simulink model "GFM_29bus"  (R2018b)
settings: Solver=ode1  StartTime=0.0  StopTime=4.5  FixedStep=Time_Step  RelTol=1e-3  EnableMultiTasking=on
PreLoadFcn:
  | Init_29bus;
InitFcn:
  | Init_29bus;
undefined symbols (not defined in the file): D1, D11, Delta, Time_Step, VSC01_Delta_P_Time_Step, VSC01_Delta_P_Value
libraries: powerlib x175, GFM_Lib x1
(part 2 of 5)

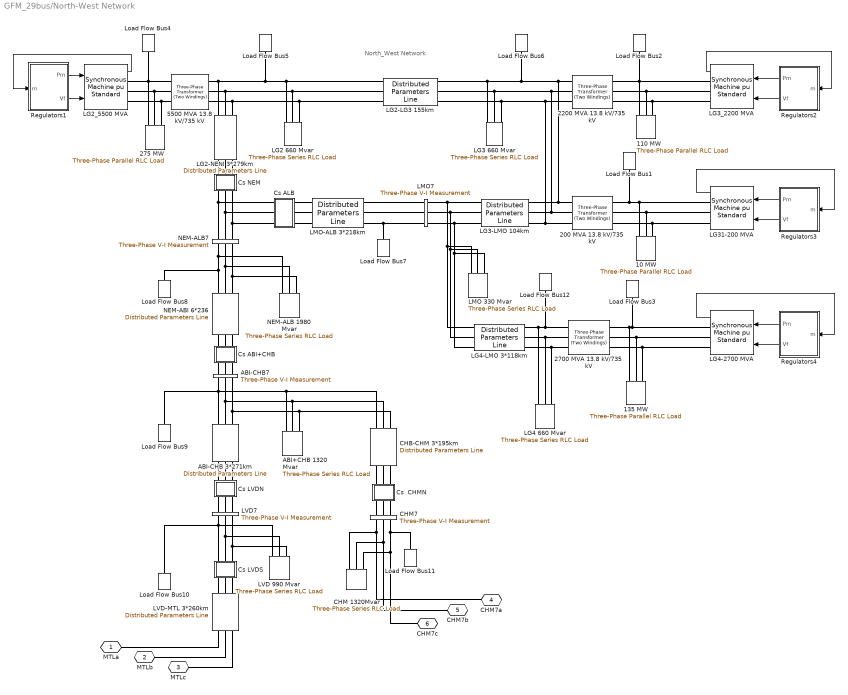
== system GFM_29bus/North-West Network ==
  note: North_West Network
  10 MW : powerlib/Elements/Three-Phase Parallel RLC Load  LConnTagsString=A|B|C  Configuration=Y (grounded)  NominalVoltage=(13800)*1  Vabc=[1e3 1e3 1e3]  Vabcp=[1e3 1e3 1e3]  NominalFrequency=60  UnbalancedPower=off  ActivePower=10000000  InductivePower=0  CapacitivePower=0  Pabc=[10e3 9e3 11e3]  QLabc=[100 90 110]  QCabc=[100 90 110]  Pabcp=[10e3 9e3 11e3]  QLabcp=[100 90 110]  QCabcp=[100 90 110]  Measurements=None  LoadType=constant PQ
  110 MW : powerlib/Elements/Three-Phase Parallel RLC Load  LConnTagsString=A|B|C  Configuration=Y (grounded)  NominalVoltage=(13800)*1  Vabc=[1e3 1e3 1e3]  Vabcp=[1e3 1e3 1e3]  NominalFrequency=60  UnbalancedPower=off  ActivePower=110000000  InductivePower=0  CapacitivePower=0  Pabc=[10e3 9e3 11e3]  QLabc=[100 90 110]  QCabc=[100 90 110]  Pabcp=[10e3 9e3 11e3]  QLabcp=[100 90 110]  QCabcp=[100 90 110]  Measurements=None  LoadType=constant PQ
  135 MW : powerlib/Elements/Three-Phase Parallel RLC Load  LConnTagsString=A|B|C  Configuration=Y (grounded)  NominalVoltage=(13800)*1  Vabc=[1e3 1e3 1e3]  Vabcp=[1e3 1e3 1e3]  NominalFrequency=60  UnbalancedPower=off  ActivePower=135000000  InductivePower=0  CapacitivePower=0  Pabc=[10e3 9e3 11e3]  QLabc=[100 90 110]  QCabc=[100 90 110]  Pabcp=[10e3 9e3 11e3]  QLabcp=[100 90 110]  QCabcp=[100 90 110]  Measurements=None  LoadType=constant PQ
  200 MVA 13.8 kV/735 kV : powerlib/Elements/Three-Phase Transformer (Two Windings)  Winding1Connection=Delta (D1)  Winding2Connection=Yg  CoreType=Three single-phase transformers  SetSaturation=off  Hysteresis=off  DataFile='basic_model'  SetInitialFlux=off  Measurements=None  UNITS=pu  NominalPower=[ 200e6 60 ]  Winding1="[ 13.8e3 0.002  0.0]"  Winding2=[ 735e3 0.002 0.12]  Rm=500  Lm=500  L0=0.5  Saturation="[ 0,0  ;  0.005,1.2  ;  1.0,1.4 ]"  InitialFluxes=[ 0.8 , -0.8 , 0.7 ]  BreakLoop=off  DiscreteSolver=Trapezoidal iterative  DataType=off  TransfoNumber=0
  2200 MVA 13.8 kV/735 kV : powerlib/Elements/Three-Phase Transformer (Two Windings)  Winding1Connection=Delta (D1)  Winding2Connection=Yg  CoreType=Three single-phase transformers  SetSaturation=off  Hysteresis=off  DataFile='basic_model'  SetInitialFlux=off  Measurements=None  UNITS=pu  NominalPower=[ 2200e6 60 ]  Winding1="[ 13.8e3 0.002  0.0]"  Winding2=[ 735e3 0.002 0.12]  Rm=500  Lm=500  L0=0.5  Saturation="[ 0,0  ;  0.005,1.2  ;  1.0,1.4 ]"  InitialFluxes=[ 0.8 , -0.8 , 0.7 ]  BreakLoop=off  DiscreteSolver=Trapezoidal iterative  DataType=off  TransfoNumber=0
  2700 MVA 13.8 kV/735 kV : powerlib/Elements/Three-Phase Transformer (Two Windings)  Winding1Connection=Delta (D1)  Winding2Connection=Yg  CoreType=Three single-phase transformers  SetSaturation=off  Hysteresis=off  DataFile='basic_model'  SetInitialFlux=off  Measurements=None  UNITS=pu  NominalPower=[ 2700e6 60 ]  Winding1="[ 13.8e3 0.002  0.0]"  Winding2=[ 735e3 0.002 0.12]  Rm=500  Lm=500  L0=0.5  Saturation="[ 0,0  ;  0.005,1.2  ;  1.0,1.4 ]"  InitialFluxes=[ 0.8 , -0.8 , 0.7 ]  BreakLoop=off  DiscreteSolver=Trapezoidal iterative  DataType=off  TransfoNumber=0
  275 MW : powerlib/Elements/Three-Phase Parallel RLC Load  LConnTagsString=A|B|C  Configuration=Y (grounded)  NominalVoltage=(13800)*1  Vabc=[1e3 1e3 1e3]  Vabcp=[1e3 1e3 1e3]  NominalFrequency=60  UnbalancedPower=off  ActivePower=275000000  InductivePower=0  CapacitivePower=0  Pabc=[10e3 9e3 11e3]  QLabc=[100 90 110]  QCabc=[100 90 110]  Pabcp=[10e3 9e3 11e3]  QLabcp=[100 90 110]  QCabcp=[100 90 110]  Measurements=None  LoadType=constant PQ
  5500 MVA 13.8 kV/735 kV : powerlib/Elements/Three-Phase Transformer (Two Windings)  Winding1Connection=Delta (D1)  Winding2Connection=Yg  CoreType=Three single-phase transformers  SetSaturation=off  Hysteresis=off  DataFile='basic_model'  SetInitialFlux=off  Measurements=None  UNITS=pu  NominalPower=[ 5500e6 60 ]  Winding1="[ 13.8e3 0.002  0.0]"  Winding2=[ 735e3 0.002 0.12]  Rm=500  Lm=500  L0=0.5  Saturation="[ 0,0  ;  0.005,1.2  ;  1.0,1.4 ]"  InitialFluxes=[ 0.8 , -0.8 , 0.7 ]  BreakLoop=off  DiscreteSolver=Trapezoidal iterative  DataType=off  TransfoNumber=0
  ABI+CHB 1320 Mvar : powerlib/Elements/Three-Phase Series RLC Load  LConnTagsString=A|B|C  Configuration=Y (grounded)  NominalVoltage=735e3  Vabc=[1e3 1e3 1e3]  Vabcp=[1e3 1e3 1e3]  NominalFrequency=60  UnbalancedPower=off  ActivePower=4400000  InductivePower=1320e6  CapacitivePower=0  Pabc=[10e3 9e3 11e3]  QLabc=[100 90 110]  QCabc=[100 90 110]  Pabcp=[10e3 9e3 11e3]  QLabcp=[100 90 110]  QCabcp=[100 90 110]  Measurements=None  LoadType=constant Z
  ABI-CHB 3*271km : powerlib/Elements/Distributed Parameters Line  Phases=3  Length=271  Frequency=60  Resistance="[0.01273  0.3864]/3"  Inductance="[0.9337e-3  4.1264e-3]/3"  Capacitance=[12.74e-9 7.751e-9]*3  x1=[-0.00156 -3.96687684446933e-08 0 0;-0.00152 -3.91975334867025e-08 0 0;-0.00148 -3.87173853476219e-08 0 0;-0.00144 -3.82284332089978e-08 0 0;-0.0014 -3.773078825433e-08 0 0;-0.00136 -3.72245636437896e-08 0 0;-0.00132 -3.67098744884875e-08 0 0;-0.00128 -3.61868378242992e-08 0 0;-0.00124 -3.56555725852517e-08 0 0;-0.0012 -3.51161995764789e-08 0 0;-0.00116 -3.45688414467516e-08 0 0;-0.00112 -3.40136226605882e-08 0 0;-0.00108 -3.34506694699529e-08 0 0;-0.00104 -3.28801098855464e-08 0 0;-0.001 -3.23020736476978e-08 0 0;-0.00096 -3.17166921968631e-08 187821.103557323 -755234.225715977;-0.00092 -3.11240986437358e-08 199188.008257712 -752316.171268998;-0.00088 -3.05244277389798e-08 210509.619322748 -749227.046612372;-0.00084 -2.99178158425874e-08 221783.362315707 -745967.554186405;-0.0008 -2.93044008928726e-08 233006.673684654 -742538.435171566;-0.00076 -2.86843223751052e-08 244177.00134537 -738940.469319947;-0.00072 -2.80577212897927e-08 255291.805261672 -735174.474777957;-0.00068 -2.74247401206185e-08 266348.558023 -731241.307900276;-0.00064 -2.67855228020416e-08 277344.745419126 -727141.863055136;-0.0006 -2.61402146865681e-08 288277.867011863 -722877.072420941;-0.00056 -2.54889625116985e-08 299145.436703644 -718447.905774304;-0.00052 -2.48319143665612e-08 309944.983302838 -713855.370269525;-0.00048 -2.41692196582383e-08 320674.051085682 -709100.510209573;-0.00044 -2.35010290777915e-08 331330.200354684 -704184.406808622;-0.0004 -2.28274945659967e-08 341911.007993395 -699108.17794619;-0.00036 -2.21487692787935e-08 352414.068017403 -693872.977912945;-0.00032 -2.14650075524591e-08 362836.992121434 -688479.997148229;-0.00028 -2.07763648685137e-08 373177.410222429 -682930.46196936;-0.00024 -2.00829978183649e-08 383432.970998484 -677225.63429278;-0.0002 -1.93850640677006e-08 393601.34242352 -671366.811347108;-0.00016 -1.8682722320637e-08 403680.212297562 -665355.325378155;-0.00012 -1.79761322836306e-08 413667.288772517 -659192.543345992;-8e-05 -1.72654546291625e-08 423560.300873321 -652879.866614107;-4e-05 -1.65508509592027e-08 433356.999014334 -646418.730630749]  x2=[-0.00156 -8.24539782860375e-08 0 0;-0.00152 -8.14137848863291e-08 0 0;-0.00148 -8.03550786940201e-08 0 0;-0.00144 -7.92781004497688e-08 0 0;-0.0014 -7.81830950491404e-08 0 0;-0.00136 -7.70703114869202e-08 0 0;-0.00132 -7.59400028004939e-08 0 0;-0.00128 -7.47924260123094e-08 0 0;-0.00124 -7.36278420714322e-08 0 0;-0.0012 -7.24465157942074e-08 0 0;-0.00116 -7.12487158040431e-08 0 0;-0.00112 -7.00347144703277e-08 0 0;-0.00108 -6.88047878464955e-08 0 0;-0.00104 -6.75592156072541e-08 0 0;-0.001 -6.62982809849896e-08 0 0;-0.00096 -6.50222707053611e-08 -41956.1732739779 -761002.997662075;-0.00092 -6.37314749221023e-08 -30476.1660907915 -761549.111628015;-0.00088 -6.24261871510431e-08 -18989.2288902512 -761922.055893291;-0.00084 -6.11067042033663e-08 -7497.97370281746 -762121.745653593;-0.0008 -5.97733261181154e-08 3994.98645917652 -762148.135501191;-0.00076 -5.84263560939685e-08 15487.0381957011 -762001.219435262;-0.00072 -5.70661004202932e-08 26975.5683132944 -761681.030863252;-0.00068 -5.56928684074994e-08 38457.9644192806 -761187.642593282;-0.00064 -5.43069723167046e-08 49931.6155158053 -760521.166817588;-0.0006 -5.29087272887284e-08 61393.9125935536 -759681.755087015;-0.00056 -5.14984512724322e-08 72842.2492250167 -758669.598276551;-0.00052 -5.00764649524203e-08 84274.0221571708 -757484.926541928;-0.00048 -4.86430916761193e-08 95686.6319034346 -756128.00926728;-0.00044 -4.71986573802513e-08 107077.48333477 -754599.155003896;-0.0004 -4.57434905167189e-08 118443.986269792 -752898.71140005;-0.00036 -4.42779219779181e-08 129783.556063753 -751027.065121953;-0.00032 -4.2802285021496e-08 141093.614196272 -748984.641765829;-0.00028 -4.13169151945712e-08 152371.588857661 -746771.905761136;-0.00024 -3.98221502574331e-08 163614.915533741 -744389.360264959;-0.0002 -3.83183301067381e-08 174821.037588984 -741837.547047599;-0.00016 -3.680579669822e-08 185987.406847871 -739117.046369375;-0.00012 -3.52848939689323e-08 197111.484174328 -736228.47684868;-8e-05 -3.37559677590401e-08 208190.740049101 -733172.495321314;-4e-05 -3.22193657331786e-08 219222.655144948 -729949.796691121]  x3=[-0.00156 -4.97060323713084e-10 0 0;-0.00152 -4.99355267685027e-10 0 0;-0.00148 -5.01536662575356e-10 0 0;-0.00144 -5.03604012353683e-10 0 0;-0.0014 -5.05556846922497e-10 0 0;-0.00136 -5.07394722224057e-10 0 0;-0.00132 -5.09117220341369e-10 0 0;-0.00128 -5.10723949593215e-10 0 0;-0.00124 -5.1221454462322e-10 0 0;-0.0012 -5.13588666482928e-10 0 0;-0.00116 -5.14846002708877e-10 0 0;-0.00112 -5.15986267393653e-10 0 0;-0.00108 -5.170092012509e-10 0 0;-0.00104 -5.1791457167428e-10 0 0;-0.001 -5.18702172790366e-10 0 0;-0.00096 -5.19371825505456e-10 139.184757397711 -1341.52529810437;-0.00092 -5.19923377546299e-10 159.398007251781 -1339.2740416806;-0.00088 -5.20356703494716e-10 179.575011373592 -1336.71824588915;-0.00084 -5.20671704816123e-10 199.711181686405 -1333.85849189596;-0.0008 -5.20868309881937e-10 219.801939398739 -1330.69542998441;-0.00076 -5.2094647398586e-10 239.842716045545 -1327.22977940752;-0.00072 -5.2090617935405e-10 259.828954527038 -1323.46232822433;-0.00068 -5.20747435149159e-10 279.75611014494 -1319.39393312075;-0.00064 -5.20470277468249e-10 299.61965163591 -1315.02551921475;-0.0006 -5.20074769334587e-10 319.415062201907 -1310.35807984598;-0.00056 -5.19561000683313e-10 339.137840537278 -1305.3926763499;-0.00052 -5.18929088340986e-10 358.783501852311 -1300.13043781644;-0.00048 -5.18179175999025e-10 378.34757889304 -1294.57256083327;-0.00044 -5.17311434181028e-10 397.825622957059 -1288.72030921369;-0.0004 -5.16326060204003e-10 417.213204905119 -1282.57501370924;-0.00036 -5.15223278133493e-10 436.505916168278 -1276.13807170713;-0.00032 -5.14003338732632e-10 455.699369750367 -1269.41094691246;-0.00028 -5.12666519405119e-10 474.789201225558 -1262.3951690154;-0.00024 -5.11213124132141e-10 493.771069730799 -1255.09233334333;-0.0002 -5.0964348340325e-10 512.640658952883 -1247.50410049812;-0.00016 -5.07957954141212e-10 531.393678109946 -1239.63219597847;-0.00012 -5.06156919620844e-10 550.02586292715 -1231.47840978759;-8e-05 -5.04240789381866e-10 568.532976606346 -1223.04459602614;-4e-05 -5.0220999913577e-10 586.910810789482 -1214.33267247064]  x4=[-0.00156 -7.23499245139953e-11 0 0;-0.00152 -6.66102552922797e-11 0 0;-0.00148 -6.08554394729331e-11 0 0;-0.00144 -5.50867856514452e-11 0 0;-0.0014 -4.93056055699484e-11 0 0;-0.00136 -4.35132138189384e-11 0 0;-0.00132 -3.7710927538348e-11 0 0;-0.00128 -3.19000661180405e-11 0 0;-0.00124 -2.60819508977922e-11 0 0;-0.0012 -2.0257904866831e-11 0 0;-0.00116 -1.44292523629998e-11 0 0;-0.00112 -8.59731877161376e-12 0 0;-0.00108 -2.76343022407925e-12 0 0;-0.00104 3.07108670365746e-12 0 0;-0.001 8.90490529276171e-12 0 0;-0.00096 1.4736698983195e-11 -1510.56660851053 -15585.3215951668;-0.00092 2.05651416753633e-11 -1275.38237576371 -15606.3269526567;-0.00088 2.63889080316609e-11 -1039.90813206307 -15623.7835659808;-0.00084 3.22066737778404e-11 -804.197422220979 -15637.6874656559;-0.0008 3.80171160041413e-11 -568.303844820181 -15648.0354900548;-0.00076 4.38189134661086e-11 -332.281040025915 -15654.8252861263;-0.00072 4.96107468850318e-11 -96.1826773886164 -15658.0553099292;-0.00068 5.53912992479382e-11 139.937556360077 -15657.7248269839;-0.00064 6.11592561070699e-11 376.025969515224 -15653.8339124394;-0.0006 6.69133058787778e-11 612.028877607613 -15646.3834510561;-0.00056 7.26521401417647e-11 847.892615611145 -15635.3751370047;-0.00052 7.83744539346086e-11 1083.5635501458 -15620.8114734809;-0.00048 8.40789460525004e-11 1318.98809167341 -15602.6957721362;-0.00044 8.97643193431258e-11 1554.11270668344 -15581.0321523248;-0.0004 9.5429281001627e-11 1788.88392986607 -15555.8255401671;-0.00036 1.01072542864576e-10 2023.24837626972 -15527.0816674293;-0.00032 1.06692821702889e-10 2257.15275344037 -15494.8070702201;-0.00028 1.12288839513627e-10 2490.54387353973 -15459.0090875047;-0.00024 1.17859323810598e-10 2723.36866543979 -15419.6958594356;-0.0002 1.23403007913709e-10 2955.57418679066 -15376.8763255019;-0.00016 1.28918631237003e-10 3187.10763605924 -15330.5602224963;-0.00012 1.34404939575301e-10 3417.91636453582 -15280.7580823012;-8e-05 1.39860685389398e-10 3647.94788830597 -15227.4812294938;-4e-05 1.45284628089745e-10 3877.14990018487 -15170.7417787711]  x5=0.00153261764655846  V1=ones(3,3)  V2=ones(3,3)  I1=ones(3,3)  I2=ones(3,3)  nHarmo=1  Measurements=None  Decoupling=off  VsMag0=0  VrMag0=0  VsAngle0=0  VrAngle0=0  IsMag0=0  IrMag0=0  IsAngle0=0  IrAngle0=0
      settings: AttributesFormatString=\n
  ABI-CHB7 : powerlib/Measurements/Three-Phase V-I Measurement  VoltageMeasurement=no  SetLabelV=on  LabelV=Vabc_ABI7  Vpu=on  VpuLL=off  CurrentMeasurement=no  SetLabelI=off  LabelI=A1  Ipu=off  Pbase=100e6  Vbase=500e3  OutputType=Magnitude  PhasorSimulation=off  PSBequivalent=0
  CHB-CHM 3*195km : powerlib/Elements/Distributed Parameters Line  Phases=3  Length=195  Frequency=60  Resistance="[0.01273  0.3864]/3"  Inductance="[0.9337e-3  4.1264e-3]/3"  Capacitance=[12.74e-9 7.751e-9]*3  x1=[-0.00112 -3.40136226605882e-08 0 0;-0.00108 -3.34506694699529e-08 0 0;-0.00104 -3.28801098855464e-08 0 0;-0.001 -3.23020736476978e-08 0 0;-0.00096 -3.17166921968631e-08 0 0;-0.00092 -3.11240986437358e-08 0 0;-0.00088 -3.05244277389798e-08 0 0;-0.00084 -2.99178158425874e-08 0 0;-0.0008 -2.93044008928726e-08 0 0;-0.00076 -2.86843223751052e-08 0 0;-0.00072 -2.80577212897927e-08 0 0;-0.00068 -2.74247401206185e-08 266348.558023 -731241.307900276;-0.00064 -2.67855228020416e-08 277344.745419126 -727141.863055136;-0.0006 -2.61402146865681e-08 288277.867011863 -722877.072420941;-0.00056 -2.54889625116985e-08 299145.436703644 -718447.905774304;-0.00052 -2.48319143665612e-08 309944.983302838 -713855.370269525;-0.00048 -2.41692196582383e-08 320674.051085682 -709100.510209573;-0.00044 -2.35010290777915e-08 331330.200354684 -704184.406808622;-0.0004 -2.28274945659967e-08 341911.007993395 -699108.17794619;-0.00036 -2.21487692787935e-08 352414.068017403 -693872.977912945;-0.00032 -2.14650075524591e-08 362836.992121434 -688479.997148229;-0.00028 -2.07763648685137e-08 373177.410222429 -682930.46196936;-0.00024 -2.00829978183649e-08 383432.970998484 -677225.63429278;-0.0002 -1.93850640677006e-08 393601.34242352 -671366.811347108;-0.00016 -1.8682722320637e-08 403680.212297562 -665355.325378155;-0.00012 -1.79761322836306e-08 413667.288772517 -659192.543345992;-8e-05 -1.72654546291625e-08 423560.300873321 -652879.866614107;-4e-05 -1.65508509592027e-08 433356.999014334 -646418.730630749]  x2=[-0.00112 -2.2052791971615e-08 0 0;-0.00108 -2.16420683624788e-08 0 0;-0.00104 -2.12264235336303e-08 0 0;-0.001 -2.08059519991191e-08 0 0;-0.00096 -2.03807493705462e-08 0 0;-0.00092 -1.99509123353226e-08 0 0;-0.00088 -1.95165386346832e-08 0 0;-0.00084 -1.90777270414618e-08 0 0;-0.0008 -1.86345773376304e-08 0 0;-0.00076 -1.81871902916102e-08 0 0;-0.00072 -1.77356676353574e-08 0 0;-0.00068 -1.72801120412301e-08 189054.242567797 -739105.585396465;-0.00064 -1.68206270986421e-08 200177.800883661 -736170.765273225;-0.0006 -1.63573172905067e-08 211255.840493863 -733068.546266429;-0.00056 -1.58902879694789e-08 222285.84234773 -729799.633793925;-0.00052 -1.54196453339989e-08 233265.298317959 -726364.771178221;-0.00048 -1.49454964041433e-08 244191.711770944 -722764.739477454;-0.00044 -1.44679489972898e-08 255062.598134493 -719000.357307787;-0.0004 -1.39871117036007e-08 265875.485462792 -715072.480657264;-0.00036 -1.35030938613299e-08 276627.914998509 -710982.002691161;-0.00032 -1.30160055319607e-08 287317.441731892 -706729.853548894;-0.00028 -1.25259574751788e-08 297941.634956747 -702317.000132509;-0.00024 -1.20330611236863e-08 308498.078823151 -697744.445886818;-0.0002 -1.1537428557863e-08 318984.372886805 -693013.230571223;-0.00016 -1.10391724802802e-08 329398.132654868 -688124.430023288;-0.00012 -1.05384061900731e-08 339736.990128175 -683079.155914099;-8e-05 -1.00352435571778e-08 349998.594339693 -677878.555495478;-4e-05 -9.52979899643775e-09 360180.611889118 -672523.811339114]  x3=[-0.00112 -4.51346938208632e-11 0 0;-0.00108 -4.21049821896206e-11 0 0;-0.00104 -3.90656962485261e-11 0 0;-0.001 -3.60175271049928e-11 0 0;-0.00096 -3.29611678863978e-11 0 0;-0.00092 -2.98973135824704e-11 0 0;-0.00088 -2.68266608872578e-11 0 0;-0.00084 -2.37499080407027e-11 0 0;-0.0008 -2.06677546698697e-11 0 0;-0.00076 -1.75809016298559e-11 0 0;-0.00072 -1.44900508444226e-11 0 0;-0.00068 -1.13959051463842e-11 1436.63532489199 -5039.5712074965;-0.00064 -8.29916811778968e-12 1512.46399636275 -5017.33500426099;-0.0006 -5.2005439299341e-12 1587.94874656368 -4993.95790231317;-0.00056 -2.10073718323644e-12 1663.07241091352 -4969.44521740442;-0.00052 9.99547252980699e-13 1737.81790693885 -4943.8025235079;-0.00048 4.09960440077225e-12 1812.16823815844 -4917.03565155107;-0.00044 7.19872933387654e-12 1886.10649794815 -4889.15068808979;-0.0004 1.02962173380095e-11 1959.61587338531 -4860.15397392427;-0.00036 1.33913640711106e-11 2032.67964907188 -4830.05210265727;-0.00032 1.64834657235041e-11 2105.28121093533 -4798.85191919472;-0.00028 1.95718191779395e-11 2177.40405000658 -4766.56051818929;-0.00024 2.2655722169474e-11 2249.031766174 -4733.18524242708;-0.0002 2.57344734451617e-11 2320.14807191261 -4698.73368115799;-0.00016 2.88073729235127e-11 2390.73679598777 -4663.21366836997;-0.00012 3.18737218536851e-11 2460.78188713236 -4626.6332810076;-8e-05 3.49328229743752e-11 2530.2674176967 -4589.00083713551;-4e-05 3.79839806723688e-11 2599.17758727035 -4550.32489404692]  x4=[-0.00112 -2.24971038730357e-10 0 0;-0.00108 -2.24970289807423e-10 0 0;-0.00104 -2.24918384580647e-10 0 0;-0.001 -2.24815334852831e-10 0 0;-0.00096 -2.24661164056595e-10 0 0;-0.00092 -2.24455907249047e-10 0 0;-0.00088 -2.24199611103816e-10 0 0;-0.00084 -2.23892333900435e-10 0 0;-0.0008 -2.23534145511091e-10 0 0;-0.00076 -2.23125127384734e-10 0 0;-0.00072 -2.22665372528558e-10 0 0;-0.00068 -2.22154985486854e-10 1507.95089400206 -11782.2652584688;-0.00064 -2.21594082317234e-10 1685.44568306095 -11758.1867357336;-0.0006 -2.2098279056424e-10 1862.55721630617 -11731.4345027329;-0.00056 -2.20321249230347e-10 2039.24522010242 -11702.0146426938;-0.00052 -2.19609608744348e-10 2215.46951712132 -11669.9338454389;-0.00048 -2.18848030927153e-10 2391.19003547742 -11635.1994058648;-0.00044 -2.1803668895499e-10 2566.36681784019 -11597.8192222834;-0.0004 -2.17175767320028e-10 2740.96003052 -11557.8017946263;-0.00036 -2.1626546178842e-10 2914.9299725259 -11515.1562225112;-0.00032 -2.15305979355796e-10 3088.23708459333 -11469.8922031737;-0.00028 -2.14297538200187e-10 3260.84195817954 -11422.0200292613;-0.00024 -2.13240367632413e-10 3432.70534442477 -11371.5505864935;-0.0002 -2.12134708043947e-10 3603.78816307707 -11318.4953511865;-0.00016 -2.10980810852243e-10 3774.05151137883 -11262.8663876431;-0.00012 -2.09778938443573e-10 3943.45667291294 -11204.67634541;-8e-05 -2.08529364113357e-10 4111.96512640654 -11143.938456401;-4e-05 -2.07232372004022e-10 4279.53855449048 -11080.6665318882]  x5=0.0011028060556417  V1=ones(3,3)  V2=ones(3,3)  I1=ones(3,3)  I2=ones(3,3)  nHarmo=1  Measurements=None  Decoupling=off  VsMag0=0  VrMag0=0  VsAngle0=0  VrAngle0=0  IsMag0=0  IrMag0=0  IsAngle0=0  IrAngle0=0
      settings: AttributesFormatString=\n
  CHM 1320Mvar : powerlib/Elements/Three-Phase Series RLC Load  LConnTagsString=A|B|C  Configuration=Y (grounded)  NominalVoltage=735e3  Vabc=[1e3 1e3 1e3]  Vabcp=[1e3 1e3 1e3]  NominalFrequency=60  UnbalancedPower=off  ActivePower=4400000  InductivePower=1320e6  CapacitivePower=0  Pabc=[10e3 9e3 11e3]  QLabc=[100 90 110]  QCabc=[100 90 110]  Pabcp=[10e3 9e3 11e3]  QLabcp=[100 90 110]  QCabcp=[100 90 110]  Measurements=None  LoadType=constant Z
  CHM7 : powerlib/Measurements/Three-Phase V-I Measurement  VoltageMeasurement=no  SetLabelV=on  LabelV=Vabc_CHM7  Vpu=on  VpuLL=off  CurrentMeasurement=no  SetLabelI=off  LabelI=A1  Ipu=off  Pbase=100e6  Vbase=735e3  OutputType=Magnitude  PhasorSimulation=off  PSBequivalent=0
  "Cs  CHMN " : Subsystem  mask{Xc=25/3}
      mask prompts: Xc "Condensator Reactance at  60Hz  (ohm):"
      mask help: Series Compensation
      mask init:
      | Cs=1/Xc/(2*pi*60);
      mask Display: disp('Cs')
  "Cs ABI+CHB " : Subsystem  mask{Xc=25/6}
      mask prompts: Xc "Condensator Reactance at  60Hz  (ohm):"
      mask help: Series Compensation
      mask init:
      | Cs=1/Xc/(2*pi*60);
      mask Display: disp('Cs')
  Cs ALB : Subsystem  mask{Xc=16/3}
      mask prompts: Xc "Reactance @ 60Hz du condensateur (ohm):"
      mask init:
      | Cs=1/Xc/(2*pi*60);
      mask Display: disp('Cs')
  "Cs LVDN " : Subsystem  mask{Xc=34/3}
      mask prompts: Xc "Condensator Reactance at  60Hz  (ohm):"
      mask help: Series Compensation
      mask init:
      | Cs=1/Xc/(2*pi*60);
      mask Display: disp('Cs')
  "Cs LVDS " : Subsystem  mask{Xc=34/3}
      mask prompts: Xc "Condensator Reactance at  60Hz  (ohm):"
      mask help: Series Compensation
      mask init:
      | Cs=1/Xc/(2*pi*60);
      mask Display: disp('Cs')
  "Cs NEM " : Subsystem  mask{Xc=16/3}
      mask prompts: Xc "Condensator Reactance at  60Hz  (ohm):"
      mask help: Series Compensation
      mask init:
      | Cs=1/Xc/(2*pi*60);
      mask Display: disp('Cs')
  LG2 660 Mvar : powerlib/Elements/Three-Phase Series RLC Load  LConnTagsString=A|B|C  Configuration=Y (grounded)  NominalVoltage=735e3  Vabc=[1e3 1e3 1e3]  Vabcp=[1e3 1e3 1e3]  NominalFrequency=60  UnbalancedPower=off  ActivePower=2200000  InductivePower=660e6  CapacitivePower=0  Pabc=[10e3 9e3 11e3]  QLabc=[100 90 110]  QCabc=[100 90 110]  Pabcp=[10e3 9e3 11e3]  QLabcp=[100 90 110]  QCabcp=[100 90 110]  Measurements=None  LoadType=constant Z
  LG2-LG3 155km : powerlib/Elements/Distributed Parameters Line  Phases=3  Length=155  Frequency=60  Resistance="[0.01273  0.3864]"  Inductance="[0.9337e-3  4.1264e-3]"  Capacitance=[12.74e-9 7.751e-9]  x1=[-0.00088 -2.46870498089306e-09 432967.319119817 -601760.567731855;-0.00084 -2.4236910908169e-09 441992.1177872 -595163.398551982;-0.0008 -2.37812607428771e-09 450916.411258577 -588430.89434775;-0.00076 -2.33202029239731e-09 459738.17022657 -581564.586032555;-0.00072 -2.28538422920291e-09 468455.388699268 -574566.034945695;-0.00068 -2.2382284893431e-09 477066.084456362 -567436.832497335;-0.00064 -2.19056379562648e-09 485568.299499894 -560178.599806632;-0.0006 -2.14240098659334e-09 493960.100499482 -552792.987333108;-0.00056 -2.09375101405114e-09 502239.579231947 -545281.674501348;-0.00052 -2.04462494058408e-09 510404.853015224 -537646.369319115;-0.00048 -1.99503393703763e-09 518454.06513647 -529888.807988964;-0.00044 -1.94498927997833e-09 526385.385274261 -522010.754513442;-0.0004 -1.89450234912964e-09 534197.009914795 -514014.000293973;-0.00036 -1.84358462478425e-09 541887.162761993 -505900.363723505;-0.00032 -1.79224768519358e-09 549454.095141415 -497671.689773026;-0.00028 -1.74050320393498e-09 556896.086397892 -489329.84957203;-0.00024 -1.68836294725727e-09 564211.44428679 -480876.739983042;-0.0002 -1.63583877140518e-09 571398.505358808 -472314.283170286;-0.00016 -1.58294261992334e-09 578455.63533824 -463644.426162603;-0.00012 -1.52968652094044e-09 585381.229494584 -454869.140410709;-8e-05 -1.47608258443414e-09 592173.713007454 -445990.42133891;-4e-05 -1.42214299947733e-09 598831.541324674 -437010.287891357]  x2=[-0.00088 -9.77818774096488e-10 445023.73878971 -584526.591412552;-0.00084 -9.6050679070525e-10 453787.292631294 -577749.57858463;-0.0008 -9.42976396352864e-10 462447.659155828 -570841.190484839;-0.00076 -9.2523157729983e-10 471002.869070649 -563802.998021056;-0.00072 -9.07276368564974e-10 479450.976994799 -556636.601617554;-0.00068 -8.89114853007925e-10 487790.061901389 -549343.630851073;-0.00064 -8.70751160400702e-10 496018.227554425 -541925.744080274;-0.0006 -8.52189466488643e-10 504133.602939995 -534384.62806864;-0.00056 -8.33433992040872e-10 512134.342691719 -526721.99760092;-0.00052 -8.1448900189054e-10 520018.627510373 -518939.595093203;-0.00048 -7.95358803965032e-10 527784.664577582 -511039.190196705;-0.00044 -7.76047748306385e-10 535430.687963486 -503022.579395372;-0.0004 -7.56560226082124e-10 542954.959028305 -494891.585597366;-0.00036 -7.36900668586749e-10 550355.766817685 -486648.057720558;-0.00032 -7.17073546234098e-10 557631.428451757 -478293.870272098;-0.00028 -6.97083367540812e-10 564780.289507808 -469830.92292217;-0.00024 -6.76934678101139e-10 571800.724396482 -461261.140072018;-0.0002 -6.56632059553301e-10 578691.136731428 -452586.470416361;-0.00016 -6.36180128537675e-10 585449.959692301 -443808.88650027;-0.00012 -6.15583535647003e-10 592075.656381045 -434930.384270634;-8e-05 -5.94846964368891e-10 598566.720171371 -425952.982622295;-4e-05 -5.73975130020824e-10 604921.67505135 -416878.72293897]  x3=[-0.00088 4.31670369824933e-12 1691.04104798713 -2581.82778924969;-0.00084 4.4152064901244e-12 1729.78041093162 -2556.03490983374;-0.0008 4.51270530211874e-12 1768.12643672765 -2529.66081012159;-0.00076 4.60917796384329e-12 1806.07040581965 -2502.71148735608;-0.00072 4.70460253824672e-12 1843.60369007625 -2475.19306958082;-0.00068 4.79895732660372e-12 1880.71775475228 -2447.11181424669;-0.00064 4.89222087344909e-12 1917.40416042951 -2418.47410678899;-0.0006 4.98437197145656e-12 1953.65456493564 -2389.28645917544;-0.00056 5.07538966626111e-12 1989.4607252413 -2359.55550842541;-0.00052 5.16525326122385e-12 2024.81449933443 -2329.2880151007;-0.00048 5.25394232213823e-12 2059.70784807166 -2298.49086176827;-0.00044 5.34143668187663e-12 2094.1328370064 -2267.17105143523;-0.0004 5.42771644497616e-12 2128.08163819305 -2235.33570595634;-0.00036 5.51276199216273e-12 2161.54653196696 -2202.99206441462;-0.00032 5.59655398481232e-12 2194.51990869988 -2170.14748147526;-0.00028 5.67907336934839e-12 2226.9942705303 -2136.80942571316;-0.00024 5.76030138157451e-12 2258.96223306839 -2102.98547791471;-0.0002 5.84021955094119e-12 2290.41652707513 -2068.68332935396;-0.00016 5.91880970474589e-12 2321.35000011533 -2033.91078004368;-0.00012 5.99605397226537e-12 2351.75561818397 -1998.67573696172;-8e-05 6.07193478881933e-12 2381.62646730571 -1962.98621225302;-4e-05 6.14643489976444e-12 2410.95575510706 -1926.85032140772]  x4=[-0.00088 -1.00528972699252e-11 1092.95151191299 -2102.92038476547;-0.00084 -1.00865716563435e-11 1124.53751640733 -2086.20052208695;-0.0008 -1.011795244335e-11 1155.86781076804 -2069.00627540033;-0.00076 -1.01470324952244e-11 1186.93527075636 -2051.34155452904;-0.00072 -1.01738051994137e-11 1217.7328318998 -2033.21037627826;-0.00068 -1.01982644680358e-11 1248.25349109855 -2014.61686352158;-0.00064 -1.02204047392639e-11 1278.49030821791 -1995.56524426345;-0.0006 -1.02402209785914e-11 1308.4364076664 -1976.05985067779;-0.00056 -1.02577086799762e-11 1338.08497995927 -1956.10511812291;-0.00052 -1.02728638668659e-11 1367.42928326685 -1935.70558413289;-0.00048 -1.02856830931017e-11 1396.46264494762 -1914.86588738586;-0.00044 -1.0296163443702e-11 1425.17846306551 -1893.59076664914;-0.0004 -1.03043025355256e-11 1453.57020789111 -1871.88505970171;-0.00036 -1.03100985178132e-11 1481.6314233865 -1849.75370223415;-0.00032 -1.03135500726083e-11 1509.35572867325 -1827.20172672631;-0.00028 -1.03146564150571e-11 1536.73681948344 -1804.23426130292;-0.00024 -1.0313417293587e-11 1563.76846959312 -1780.85652856756;-0.0002 -1.03098329899634e-11 1590.44453223819 -1757.07384441507;-0.00016 -1.03039043192262e-11 1616.75894151203 -1732.89161682271;-0.00012 -1.02956326295038e-11 1642.70571374491 -1708.31534462051;-8e-05 -1.02850198017072e-11 1668.27894886457 -1683.35061624082;-4e-05 -1.0272068249102e-11 1693.47283173789 -1658.0031084476]  x5=0.000876589428843401  V1=ones(3,3)  V2=ones(3,3)  I1=ones(3,3)  I2=ones(3,3)  nHarmo=1  Measurements=None  Decoupling=off  VsMag0=0  VrMag0=0  VsAngle0=0  VrAngle0=0  IsMag0=0  IrMag0=0  IsAngle0=0  IrAngle0=0
      settings: AttributesFormatString=\n
  LG2-NENI 3*279km : powerlib/Elements/Distributed Parameters Line  Phases=3  Length=279  Frequency=60  Resistance="[0.01273  0.3864]/3"  Inductance="[0.9337e-3  4.1264e-3]/3"  Capacitance=[12.74e-9 7.751e-9]*3  x1=[-0.0016 -3.17369651108322e-09 0 0;-0.00156 -3.14022097034721e-09 0 0;-0.00152 -3.10603137044265e-09 0 0;-0.00148 -3.07113548578973e-09 0 0;-0.00144 -3.03554125141168e-09 0 0;-0.0014 -2.99925676113046e-09 0 0;-0.00136 -2.96229026572624e-09 0 0;-0.00132 -2.9246501710613e-09 0 0;-0.00128 -2.88634503616857e-09 0 0;-0.00124 -2.8473835713054e-09 0 0;-0.0012 -2.80777463597289e-09 0 0;-0.00116 -2.76752723690139e-09 0 0;-0.00112 -2.72665052600236e-09 0 0;-0.00108 -2.68515379828734e-09 0 0;-0.00104 -2.64304648975437e-09 0 0;-0.001 -2.6003381752423e-09 405310.525020648 -620725.219641236;-0.00096 -2.55703856625353e-09 414624.437229961 -614542.931576135;-0.00092 -2.51315750874577e-09 423844.067417816 -608220.901747987;-0.00088 -2.46870498089306e-09 432967.319119817 -601760.567731855;-0.00084 -2.4236910908169e-09 441992.1177872 -595163.398551982;-0.0008 -2.37812607428771e-09 450916.411258577 -588430.89434775;-0.00076 -2.33202029239731e-09 459738.17022657 -581564.586032555;-0.00072 -2.28538422920291e-09 468455.388699268 -574566.034945695;-0.00068 -2.2382284893431e-09 477066.084456362 -567436.832497335;-0.00064 -2.19056379562648e-09 485568.299499894 -560178.599806633;-0.0006 -2.14240098659334e-09 493960.100499482 -552792.987333108;-0.00056 -2.09375101405114e-09 502239.579231947 -545281.674501348;-0.00052 -2.04462494058408e-09 510404.853015224 -537646.369319115;-0.00048 -1.99503393703763e-09 518454.06513647 -529888.807988964;-0.00044 -1.94498927997833e-09 526385.385274261 -522010.754513442;-0.0004 -1.89450234912964e-09 534197.009914795 -514014.000293973;-0.00036 -1.84358462478425e-09 541887.162761993 -505900.363723505;-0.00032 -1.79224768519358e-09 549454.095141415 -497671.689773026;-0.00028 -1.74050320393498e-09 556896.086397892 -489329.84957203;-0.00024 -1.68836294725727e-09 564211.44428679 -480876.739983042;-0.0002 -1.63583877140518e-09 571398.505358808 -472314.283170286;-0.00016 -1.58294261992334e-09 578455.63533824 -463644.426162603;-0.00012 -1.52968652094044e-09 585381.229494584 -454869.140410709;-8e-05 -1.47608258443414e-09 592173.713007454 -445990.42133891;-4e-05 -1.42214299947733e-09 598831.541324674 -437010.287891357]  x2=[-0.0016 -2.46236129996295e-08 0 0;-0.00156 -2.43308871432278e-08 0 0;-0.00152 -2.40326286529104e-08 0 0;-0.00148 -2.37289053500859e-08 0 0;-0.00144 -2.34197862988142e-08 0 0;-0.0014 -2.31053417901017e-08 0 0;-0.00136 -2.27856433259182e-08 0 0;-0.00132 -2.24607636029373e-08 0 0;-0.00128 -2.21307764960066e-08 0 0;-0.00124 -2.17957570413483e-08 0 0;-0.0012 -2.14557814194974e-08 0 0;-0.00116 -2.11109269379785e-08 0 0;-0.00112 -2.07612720137268e-08 0 0;-0.00108 -2.04068961552568e-08 0 0;-0.00104 -2.00478799445826e-08 0 0;-0.001 -1.96843050188946e-08 243857.082602521 -727661.340796743;-0.00096 -1.93162540519955e-08 254801.844915079 -723901.454430001;-0.00092 -1.89438107355012e-08 265688.667485421 -719976.959115181;-0.00088 -1.85670597598102e-08 276515.074743977 -715888.747248675;-0.00084 -1.81860867948453e-08 287278.604859102 -711637.748454607;-0.0008 -1.78009784705734e-08 297976.810296867 -707224.929373443;-0.00076 -1.74118223573064e-08 308607.258377612 -702651.293442187;-0.00072 -1.70187069457885e-08 319167.531829119 -697917.88066621;-0.00068 -1.66217216270741e-08 329655.229336271 -693025.767382756;-0.00064 -1.62209566722015e-08 340067.966087097 -687976.066016199;-0.0006 -1.58165032116651e-08 350403.374315057 -682769.924825083;-0.00056 -1.54084532146941e-08 360659.103837447 -677408.527641018;-0.00052 -1.49968994683389e-08 370832.822589816 -671893.093599491;-0.00048 -1.45819355563724e-08 380922.217156255 -666224.876862638;-0.00044 -1.41636558380096e-08 390924.993295445 -660405.166334065;-0.0004 -1.37421554264515e-08 400838.876462354 -654435.28536576;-0.00036 -1.33175301672566e-08 410661.612325442 -648316.591457172;-0.00032 -1.28898766165472e-08 420390.967279283 -642050.47594653;-0.00028 -1.24592920190528e-08 430024.728952461 -635638.363694466;-0.00024 -1.20258742859976e-08 439560.706710651 -629081.71276001;-0.0002 -1.15897219728364e-08 448996.732154745 -622382.014069042;-0.00016 -1.11509342568442e-08 458330.65961393 -615540.791075268;-0.00012 -1.07096109145635e-08 467560.366633594 -608559.599413801;-8e-05 -1.02658522991166e-08 476683.754457955 -601440.026547423;-4e-05 -9.81975931738582e-09 485698.748507297 -594183.691405605]  x3=[-0.0016 -1.56473012381929e-10 0 0;-0.00156 -1.58154913178634e-10 0 0;-0.00152 -1.59800850911952e-10 0 0;-0.00148 -1.61410451309836e-10 0 0;-0.00144 -1.62983348363037e-10 0 0;-0.0014 -1.64519184408328e-10 0 0;-0.00136 -1.66017610209838e-10 0 0;-0.00132 -1.67478285038462e-10 0 0;-0.00128 -1.68900876749339e-10 0 0;-0.00124 -1.70285061857382e-10 0 0;-0.0012 -1.71630525610834e-10 0 0;-0.00116 -1.72936962062842e-10 0 0;-0.00112 -1.74204074141021e-10 0 0;-0.00108 -1.75431573715012e-10 0 0;-0.00104 -1.76619181661998e-10 0 0;-0.001 -1.77766627930173e-10 -295.521587162754 -2742.85495450109;-0.00096 -1.78873651600151e-10 -254.128191861341 -2746.999265987;-0.00092 -1.79940000944296e-10 -212.677010000606 -2750.51893352893;-0.00088 -1.80965433483962e-10 -171.177467221846 -2753.41315678484;-0.00084 -1.81949716044634e-10 -129.639000163212 -2755.68127763333;-0.0008 -1.82892624808944e-10 -88.0710543138991 -2757.32278032326;-0.00076 -1.83793945367572e-10 -46.4830818663279 -2758.33729159109;-0.00072 -1.84653472767995e-10 -4.88453956679348 -2758.7245807457;-0.00068 -1.85471011561094e-10 36.7151134349161 -2758.48455972087;-0.00064 -1.86246375845597e-10 78.3064177364483 -2757.61728309532;-0.0006 -1.86979389310354e-10 119.879915833873 -2756.12294808028;-0.00056 -1.87669885274424e-10 161.426154272237 -2754.00189447463;-0.00052 -1.88317706724978e-10 202.9356857952 -2751.25460458768;-0.00048 -1.88922706353005e-10 244.399071493256 -2747.88170312946;-0.00044 -1.89484746586808e-10 285.806882950062 -2743.88395706866;-0.0004 -1.90003699623284e-10 327.149704386378 -2739.26227545828;-0.00036 -1.90479447456988e-10 368.418134801137 -2734.01770922885;-0.00032 -1.90911881906965e-10 409.602790109144 -2728.1514509495;-0.00028 -1.9130090464135e-10 450.694305274944 -2721.66483455679;-0.00024 -1.91646427199728e-10 491.683336442347 -2714.55933505133;-0.0002 -1.9194837101325e-10 532.560563059139 -2706.83656816245;-0.00016 -1.92206667422495e-10 573.316689996499 -2698.49828998073;-0.00012 -1.92421257693089e-10 613.942449662625 -2689.54639655873;-8e-05 -1.92592093029053e-10 654.428604110113 -2679.98292347981;-4e-05 -1.92719134583905e-10 694.765947136578 -2669.81004539528]  x4=[-0.0016 2.44847306854454e-11 0 0;-0.00156 2.6808792531249e-11 0 0;-0.00152 2.91267582888202e-11 0 0;-0.00148 3.14381008727351e-11 0 0;-0.00144 3.3742294703622e-11 0 0;-0.0014 3.60388158276746e-11 0 0;-0.00136 3.83271420357934e-11 0 0;-0.00132 4.06067529823325e-11 0 0;-0.00128 4.28771303034211e-11 0 0;-0.00124 4.51377577348354e-11 0 0;-0.0012 4.73881212293922e-11 0 0;-0.00116 4.96277090738392e-11 0 0;-0.00112 5.18560120052139e-11 0 0;-0.00108 5.40725233266459e-11 0 0;-0.00104 5.62767390225749e-11 0 0;-0.001 5.84681578733601e-11 4695.68217946984 -13362.2600276785;-0.00096 6.06462815692529e-11 4896.63935162447 -13289.9339141652;-0.00092 6.28106148237081e-11 5096.48307021735 -13214.5857842873;-0.00088 6.4960665486008e-11 5295.16789251027 -13136.2327715597;-0.00084 6.70959446531734e-11 5492.64863928801 -13054.892692782;-0.0008 6.92159667811353e-11 5688.88040513176 -12970.5840439865;-0.00076 7.13202497951444e-11 5883.8185686302 -12883.325996233;-0.00072 7.34083151993896e-11 6077.41880252602 -12793.138391249;-0.00068 7.54796881858049e-11 6269.63708379558 -12700.0417369182;-0.00064 7.75338977420358e-11 6460.42970365933 -12604.0572026168;-0.0006 7.95704767585441e-11 6649.75327752084 -12505.2066144004;-0.00056 8.1588962134824e-11 6837.56475483207 -12403.5124500402;-0.00052 8.35888948847077e-11 7023.8214288827 -12298.9978339121;-0.00048 8.55698202407345e-11 7208.48094651126 -12191.6865317387;-0.00044 8.75312877575613e-11 7391.50131773588 -12081.6029451845;-0.0004 8.94728514143898e-11 7572.84092530243 -11968.772106308;-0.00036 9.13940697163875e-11 7752.45853414797 -11853.2196718687;-0.00032 9.32945057950807e-11 7930.3133007772 -11734.9719174939;-0.00028 9.51737275076936e-11 8106.36478254994 -11614.0557317032;-0.00024 9.70313075354146e-11 8280.57294687744 -11490.4986097944;-0.0002 9.88668234805643e-11 8452.89818032544 -11364.3286475916;-0.00016 1.00679857962646e-10 8623.30129762193 -11235.5745350561;-0.00012 1.02469998713253e-10 8791.74355056752 -11104.2655497628;-8e-05 1.04236838669816e-10 8958.18663684648 -10970.4315502426;-4e-05 1.05979976068165e-10 9122.59270873633 -10834.1029691928]  x5=0.00157786097191812  V1=ones(3,3)  V2=ones(3,3)  I1=ones(3,3)  I2=ones(3,3)  nHarmo=1  Measurements=None  Decoupling=off  VsMag0=0  VrMag0=0  VsAngle0=0  VrAngle0=0  IsMag0=0  IrMag0=0  IsAngle0=0  IrAngle0=0
      settings: AttributesFormatString=\n
  LG2_5500 MVA : powerlib/Machines/Synchronous Machine pu Standard  PresetModel=No  MechanicalLoad=Mechanical power Pm  ShowDetailedParameters=on  RotorType=Salient-pole  Units=per unit standard parameters  MeasurementBus=off  NominalParameters="[5500E6  13800   60 ]"  Reactances1=[ 31 32 33 34 35 36 37 ]  Reactances2=[ 1.305, 0.296, 0.252, 0.474, 0.243, 0.18 ]  dAxisTimeConstants=Short-circuit  qAxisTimeConstants=Open-circuit  TimeConstants1=[]  TimeConstants2=[]  TimeConstants3=[]  TimeConstants4=[]  TimeConstants5=[ 1.01, 0.053, 0.1 ]  TimeConstants6=[]  TimeConstants7=[]  TimeConstants8=[]  StatorResistance=2.8544e-3  Mechanical="[ 4.1  0  32]"  PolePairs=32  InitialConditions=[0 -68.2322 0.822292 0.822292 0.822292 4.1842 -115.816 124.184 1.25511]  SetSaturation=off  Saturation=[0.6404,0.7127,0.8441,0.9214,0.9956,1.082,1.19,1.316,1.457;0.7,0.7698,0.8872,0.9466,0.9969,1.046,1.1,1.151,1.201]  LoadFlowParameters=[2 4000000000 0 0 0]  TsPowergui=0  TsBlock=-1  IterativeModel=Trapezoidal non iterative  IterativeDiscreteModel=Trapezoidal non iterative  BusType=swing  Pref=0  Qref=0  Qmin=-Inf  Qmax=Inf  PLF=0  QLF=0
      settings: AttributesFormatString=\n\n
  LG3 660 Mvar : powerlib/Elements/Three-Phase Series RLC Load  LConnTagsString=A|B|C  Configuration=Y (grounded)  NominalVoltage=735e3  Vabc=[1e3 1e3 1e3]  Vabcp=[1e3 1e3 1e3]  NominalFrequency=60  UnbalancedPower=off  ActivePower=2200000  InductivePower=660e6  CapacitivePower=0  Pabc=[10e3 9e3 11e3]  QLabc=[100 90 110]  QCabc=[100 90 110]  Pabcp=[10e3 9e3 11e3]  QLabcp=[100 90 110]  QCabcp=[100 90 110]  Measurements=None  LoadType=constant Z
  LG3-LMO 104km : powerlib/Elements/Distributed Parameters Line  Phases=3  Length=104  Frequency=60  Resistance="[0.01273  0.3864]"  Inductance="[0.9337e-3  4.1264e-3]"  Capacitance=[12.74e-9 7.751e-9]  x1=[-0.0006 -8.52189466488643e-10 0 0;-0.00056 -8.33433992040872e-10 0 0;-0.00052 -8.1448900189054e-10 0 0;-0.00048 -7.95358803965032e-10 0 0;-0.00044 -7.76047748306385e-10 0 0;-0.0004 -7.56560226082124e-10 0 0;-0.00036 -7.36900668586749e-10 550355.766817685 -486648.057720558;-0.00032 -7.17073546234098e-10 557631.428451757 -478293.870272098;-0.00028 -6.97083367540812e-10 564780.289507808 -469830.92292217;-0.00024 -6.76934678101139e-10 571800.724396482 -461261.140072018;-0.0002 -6.56632059553301e-10 578691.136731428 -452586.470416361;-0.00016 -6.36180128537675e-10 585449.959692301 -443808.88650027;-0.00012 -6.15583535647003e-10 592075.656381045 -434930.384270634;-8e-05 -5.94846964368891e-10 598566.720171371 -425952.982622295;-4e-05 -5.73975130020824e-10 604921.67505135 -416878.72293897]  x2=[-0.0006 -5.78031248366562e-09 0 0;-0.00056 -5.65921108704781e-09 0 0;-0.00052 -5.53682283463176e-09 0 0;-0.00048 -5.41317555645064e-09 0 0;-0.00044 -5.28829736882922e-09 0 0;-0.0004 -5.16221666799046e-09 0 0;-0.00036 -5.03496212359846e-09 509411.244984698 -556032.262755338;-0.00032 -4.90656267223922e-09 517737.812456147 -548287.595594527;-0.00028 -4.77704751084071e-09 525946.650813823 -540418.252562708;-0.00024 -4.64644609003373e-09 534035.893438675 -532426.023080625;-0.0002 -4.51478810745513e-09 542003.700906689 -524312.72451234;-0.00016 -4.38210350099476e-09 549848.261407157 -516080.201751981;-0.00012 -4.24842244198792e-09 557567.791154671 -507730.32680423;-8e-05 -4.11377532835461e-09 565160.534794736 -499264.998358643;-4e-05 -3.97819277768732e-09 572624.765802925 -490686.141357908]  x3=[-0.0006 -4.45154221739809e-11 0 0;-0.00056 -4.47725440719708e-11 0 0;-0.00052 -4.50194850795408e-11 0 0;-0.00048 -4.52561890444351e-11 0 0;-0.00044 -4.54826021422135e-11 0 0;-0.0004 -4.56986728884901e-11 0 0;-0.00036 -4.59043521506404e-11 -30.2364266514217 -878.887290252249;-0.00032 -4.60995931589738e-11 -16.9799648509832 -879.243256593737;-0.00028 -4.62843515173689e-11 -3.7196419529666 -879.399290600946;-0.00024 -4.64585852133682e-11 9.54152675955334 -879.35535679309;-0.0002 -4.66222546277318e-11 22.8005258111707 -879.111465160336;-0.00016 -4.67753225434462e-11 36.0543402198421 -878.667671161539;-0.00012 -4.69177541541874e-11 49.2999561824668 -878.024075711628;-8e-05 -4.70495170722354e-11 62.5343617602003 -877.180825158657;-4e-05 -4.7170581335839e-11 75.754547563343 -876.13811125053]  x4=[-0.0006 3.90789373635253e-11 0 0;-0.00056 3.95181428414206e-11 0 0;-0.00052 3.99483622344238e-11 0 0;-0.00048 4.03694977143549e-11 0 0;-0.00044 4.07814535186375e-11 0 0;-0.0004 4.11841359720742e-11 0 0;-0.00036 4.15774535081477e-11 3670.35195488091 -3222.9463627607;-0.00032 4.19613166898421e-11 3718.5337242689 -3167.23444298592;-0.00028 4.23356382299803e-11 3765.86993115525 -3110.80232141188;-0.00024 4.27003330110719e-11 3812.34981169475 -3053.66283021636;-0.0002 4.30553181046689e-11 3857.96279676337 -2995.82896242692;-0.00016 4.3400512790222e-11 3902.69851436165 -2937.31386896635;-0.00012 4.37358385734368e-11 3946.54679197322 -2878.1308556623;-8e-05 4.40612192041218e-11 3989.49765887785 -2818.29338022161;-4e-05 4.43765806935275e-11 4031.54134841882 -2757.81504917019]  x5=0.000588163229675572  V1=ones(3,3)  V2=ones(3,3)  I1=ones(3,3)  I2=ones(3,3)  nHarmo=1  Measurements=None  Decoupling=off  VsMag0=0  VrMag0=0  VsAngle0=0  VrAngle0=0  IsMag0=0  IrMag0=0  IsAngle0=0  IrAngle0=0
      settings: AttributesFormatString=\n
  LG31-200 MVA : powerlib/Machines/Synchronous Machine pu Standard  PresetModel=No  MechanicalLoad=Mechanical power Pm  ShowDetailedParameters=on  RotorType=Salient-pole  Units=per unit standard parameters  MeasurementBus=off  NominalParameters="[200E6  13800   60 ]"  Reactances1=[ 31 32 33 34 35 36 37 ]  Reactances2=[ 1.305, 0.296, 0.252, 0.474, 0.243, 0.18 ]  dAxisTimeConstants=Short-circuit  qAxisTimeConstants=Open-circuit  TimeConstants1=[]  TimeConstants2=[]  TimeConstants3=[]  TimeConstants4=[]  TimeConstants5=[ 1.01, 0.053, 0.1 ]  TimeConstants6=[]  TimeConstants7=[]  TimeConstants8=[]  StatorResistance=2.8544e-3  Mechanical="[ 3.2  0  32]"  PolePairs=32  InitialConditions=[0 -65.0253 0.900243 0.900243 0.900243 0.798134 -119.202 120.798 1.40505]  SetSaturation=off  Saturation=[0.6404,0.7127,0.8441,0.9214,0.9956,1.082,1.19,1.316,1.457;0.7,0.7698,0.8872,0.9466,0.9969,1.046,1.1,1.151,1.201]  LoadFlowParameters=[1 180000000 0 0 0]  TsPowergui=0  TsBlock=-1  IterativeModel=Trapezoidal non iterative  IterativeDiscreteModel=Trapezoidal non iterative  BusType=PV  Pref=180000000  Qref=0  Qmin=-Inf  Qmax=Inf  PLF=0  QLF=0
      settings: AttributesFormatString=\n\n
  LG3_2200 MVA : powerlib/Machines/Synchronous Machine pu Standard  PresetModel=No  MechanicalLoad=Mechanical power Pm  ShowDetailedParameters=on  RotorType=Salient-pole  Units=per unit standard parameters  MeasurementBus=off  NominalParameters="[2200E6  13800   60 ]"  Reactances1=[ 31 32 33 34 35 36 37 ]  Reactances2=[ 1.305, 0.296, 0.252, 0.474, 0.243, 0.18 ]  dAxisTimeConstants=Short-circuit  qAxisTimeConstants=Open-circuit  TimeConstants1=[]  TimeConstants2=[]  TimeConstants3=[]  TimeConstants4=[]  TimeConstants5=[ 1.01, 0.053, 0.1 ]  TimeConstants6=[]  TimeConstants7=[]  TimeConstants8=[]  StatorResistance=2.8544e-3  Mechanical="[ 3.2  0  32]"  PolePairs=32  InitialConditions=[0 -67.4267 0.818333 0.818333 0.818333 0.465769 -119.534 120.466 1.33761]  SetSaturation=off  Saturation=[0.6404,0.7127,0.8441,0.9214,0.9956,1.082,1.19,1.316,1.457;0.7,0.7698,0.8872,0.9466,0.9969,1.046,1.1,1.151,1.201]  LoadFlowParameters=[1 1800000000 0 0 0]  TsPowergui=0  TsBlock=-1  IterativeModel=Trapezoidal non iterative  IterativeDiscreteModel=Trapezoidal non iterative  BusType=PV  Pref=1800000000  Qref=0  Qmin=-Inf  Qmax=Inf  PLF=0  QLF=0
      settings: AttributesFormatString=\n\n
  LG4 660 Mvar : powerlib/Elements/Three-Phase Series RLC Load  LConnTagsString=A|B|C  Configuration=Y (grounded)  NominalVoltage=735e3  Vabc=[1e3 1e3 1e3]  Vabcp=[1e3 1e3 1e3]  NominalFrequency=60  UnbalancedPower=off  ActivePower=2200000  InductivePower=660e6  CapacitivePower=0  Pabc=[10e3 9e3 11e3]  QLabc=[100 90 110]  QCabc=[100 90 110]  Pabcp=[10e3 9e3 11e3]  QLabcp=[100 90 110]  QCabcp=[100 90 110]  Measurements=None  LoadType=constant Z
  LG4-2700 MVA : powerlib/Machines/Synchronous Machine pu Standard  PresetModel=No  MechanicalLoad=Mechanical power Pm  ShowDetailedParameters=on  RotorType=Salient-pole  Units=per unit standard parameters  MeasurementBus=off  NominalParameters="[2700E6  13800   60 ]"  Reactances1=[ 31 32 33 34 35 36 37 ]  Reactances2=[ 1.305, 0.296, 0.252, 0.474, 0.243, 0.18 ]  dAxisTimeConstants=Short-circuit  qAxisTimeConstants=Open-circuit  TimeConstants1=[]  TimeConstants2=[]  TimeConstants3=[]  TimeConstants4=[]  TimeConstants5=[ 1.01, 0.053, 0.1 ]  TimeConstants6=[]  TimeConstants7=[]  TimeConstants8=[]  StatorResistance=2.8544e-3  Mechanical="[ 3.7  0  32]"  PolePairs=32  InitialConditions=[0 -66.0751 0.928325 0.928325 0.928325 3.71347 -116.287 123.713 1.33221]  SetSaturation=off  Saturation=[0.6404,0.7127,0.8441,0.9214,0.9956,1.082,1.19,1.316,1.457;0.7,0.7698,0.8872,0.9466,0.9969,1.046,1.1,1.151,1.201]  LoadFlowParameters=[1 2500000000 0 0 0]  TsPowergui=0  TsBlock=-1  IterativeModel=Trapezoidal non iterative  IterativeDiscreteModel=Trapezoidal non iterative  BusType=PV  Pref=2500000000  Qref=0  Qmin=-Inf  Qmax=Inf  PLF=0  QLF=0
      settings: AttributesFormatString=\n\n
  LG4-LMO 3*118km : powerlib/Elements/Distributed Parameters Line  Phases=3  Length=118  Frequency=60  Resistance="[0.01273  0.3864]/3"  Inductance="[0.9337e-3  4.1264e-3]/3"  Capacitance=[12.74e-9 7.751e-9]*3  x1=[-0.00068 -1.68012162347326e-09 0 0;-0.00064 -1.66116500854653e-09 0 0;-0.0006 -1.64183065902213e-09 0 0;-0.00056 -1.62212297136441e-09 0 0;-0.00052 -1.6020464269316e-09 0 0;-0.00048 -1.58160559095677e-09 0 0;-0.00044 -1.56080511150973e-09 516880.954089849 -533087.859689799;-0.0004 -1.53964971844015e-09 524860.692753916 -525233.170384248;-0.00036 -1.51814422230197e-09 532721.082622658 -517259.04758517;-0.00032 -1.49629351325956e-09 540460.336311202 -509167.304539323;-0.00028 -1.47410255997572e-09 548076.69398 -500959.781239295;-0.00024 -1.45157640848186e-09 555568.423735 -492638.344005107;-0.0002 -1.42872018103057e-09 562933.82202146 -484204.885059824;-0.00016 -1.40553907493087e-09 570171.214011327 -475661.322099283;-0.00012 -1.38203836136639e-09 577278.953984075 -467009.597856026;-8e-05 -1.35822338419672e-09 584255.425700929 -458251.679657536;-4e-05 -1.3340995587423e-09 591099.042772382 -449389.558978885]  x2=[-0.00068 -6.0185448587352e-09 0 0;-0.00064 -5.90009948707195e-09 0 0;-0.0006 -5.78031248366562e-09 0 0;-0.00056 -5.65921108704781e-09 0 0;-0.00052 -5.53682283463176e-09 0 0;-0.00048 -5.41317555645064e-09 0 0;-0.00044 -5.28829736882922e-09 492412.522599082 -571140.553932508;-0.0004 -5.16221666799046e-09 500968.841789116 -563650.492974617;-0.00036 -5.03496212359846e-09 509411.244984698 -556032.262755338;-0.00032 -4.90656267223922e-09 517737.812456147 -548287.595594527;-0.00028 -4.77704751084071e-09 525946.650813823 -540418.252562708;-0.00024 -4.64644609003373e-09 534035.893438675 -532426.023080625;-0.0002 -4.51478810745513e-09 542003.700906689 -524312.72451234;-0.00016 -4.38210350099476e-09 549848.261407157 -516080.201751981;-0.00012 -4.24842244198792e-09 557567.791154671 -507730.32680423;-8e-05 -4.11377532835461e-09 565160.534794736 -499264.998358643;-4e-05 -3.97819277768732e-09 572624.765802925 -490686.141357908]  x3=[-0.00068 -1.24605101780502e-10 0 0;-0.00064 -1.25220856868755e-10 0 0;-0.0006 -1.25808137814014e-10 0 0;-0.00056 -1.26366811073658e-10 0 0;-0.00052 -1.26896749610204e-10 0 0;-0.00048 -1.273978329202e-10 0 0;-0.00044 -1.27869947061622e-10 2439.60066402425 -4653.83725506388;-0.0004 -1.28312984679786e-10 2509.49876429483 -4616.52129637602;-0.00036 -1.28726845031757e-10 2578.8262261874 -4578.15558055655;-0.00032 -1.29111434009262e-10 2647.56728523499 -4538.74883163839;-0.00028 -1.29466664160082e-10 2715.70631031356 -4498.31001037642;-0.00024 -1.29792454707945e-10 2783.22780719641 -4456.84831220987;-0.0002 -1.3008873157089e-10 2850.11642207745 -4414.37316517134;-0.00016 -1.30355427378113e-10 2916.35694506247 -4370.89422774298;-0.00012 -1.30592481485288e-10 2981.93431362776 -4326.42138666022;-8e-05 -1.30799839988355e-10 3046.83361604525 -4280.9647546636;-4e-05 -1.30977455735778e-10 3111.04009477322 -4234.53466819924]  x4=[-0.00068 8.45924509246265e-11 0 0;-0.00064 8.55355553235319e-11 0 0;-0.0006 8.6459209674784e-11 0 0;-0.00056 8.73632039473485e-11 0 0;-0.00052 8.82473325807236e-11 0 0;-0.00048 8.91113945316824e-11 0 0;-0.00044 8.99551933199886e-11 7760.49572203623 -8389.18257887061;-0.0004 9.07785370730744e-11 7886.11533320204 -8271.20760955468;-0.00036 9.15812385696706e-11 8009.94170974805 -8151.3518389562;-0.00032 9.2363115282379e-11 8131.94669462406 -8029.64252124381;-0.00028 9.31239894191777e-11 8252.10254494863 -7906.10733206677;-0.00024 9.38636879638496e-11 8370.38193831758 -7780.77436226179;-0.0002 9.45820427153245e-11 8486.75797901686 -7653.67211146536;-0.00016 9.52788903259268e-11 8601.20420413839 -7524.82948163325;-0.00012 9.59540723385191e-11 8713.69458959752 -7394.27577046838;-8e-05 9.66074352225342e-11 8824.20355605069 -7262.04066475883;-4e-05 9.72388304088868e-11 8932.7059747119 -7128.15423362728]  x5=0.000667339049054976  V1=ones(3,3)  V2=ones(3,3)  I1=ones(3,3)  I2=ones(3,3)  nHarmo=1  Measurements=None  Decoupling=off  VsMag0=0  VrMag0=0  VsAngle0=0  VrAngle0=0  IsMag0=0  IrMag0=0  IsAngle0=0  IrAngle0=0
      settings: AttributesFormatString=\n
  LMO 330 Mvar : powerlib/Elements/Three-Phase Series RLC Load  LConnTagsString=A|B|C  Configuration=Y (grounded)  NominalVoltage=735e3  Vabc=[1e3 1e3 1e3]  Vabcp=[1e3 1e3 1e3]  NominalFrequency=60  UnbalancedPower=off  ActivePower=1100000  InductivePower=330e6  CapacitivePower=0  Pabc=[10e3 9e3 11e3]  QLabc=[100 90 110]  QCabc=[100 90 110]  Pabcp=[10e3 9e3 11e3]  QLabcp=[100 90 110]  QCabcp=[100 90 110]  Measurements=None  LoadType=constant Z
  LMO-ALB 3*218km : powerlib/Elements/Distributed Parameters Line  Phases=3  Length=218  Frequency=60  Resistance="[0.01273  0.3864]/3"  Inductance="[0.9337e-3  4.1264e-3]/3"  Capacitance=[12.74e-9 7.751e-9]*3  x1=[-0.00124 -7.52141822684451e-09 300534.093454917 -691628.864422308;-0.0012 -7.4244340765829e-09 310929.078838548 -687018.443221772;-0.00116 -7.32576167403787e-09 321253.361630989 -682251.799951843;-0.00112 -7.22542345646284e-09 331504.594179366 -677330.018506093;-0.00108 -7.1234422399032e-09 341680.445441801 -672254.21805518;-0.00104 -7.01984121400817e-09 351778.601517469 -667025.552792355;-0.001 -6.9146439367576e-09 361796.766172761 -661645.211671009;-0.00096 -6.80787432910516e-09 371732.661363429 -656114.418134314;-0.00092 -6.6995566695389e-09 381584.027752588 -650434.429837024;-0.00088 -6.58971558856049e-09 391348.625224476 -644606.538359498;-0.00084 -6.47837606308453e-09 401024.233393835 -638632.068913998;-0.0008 -6.36556341075896e-09 410608.652110806 -632512.380043356;-0.00076 -6.25130328420807e-09 420099.701961226 -626248.863312047;-0.00072 -6.13562166519929e-09 429495.224762205 -619842.94298976;-0.00068 -6.0185448587352e-09 438793.084052882 -613296.075727536;-0.00064 -5.90009948707195e-09 447991.165580236 -606609.750226531;-0.0006 -5.78031248366562e-09 457087.377779848 -599785.486899504;-0.00056 -5.65921108704781e-09 466079.652251507 -592824.837525087;-0.00052 -5.53682283463176e-09 474965.944229544 -585729.384894919;-0.00048 -5.41317555645063e-09 483744.233047794 -578500.742453742;-0.00044 -5.28829736882922e-09 492412.522599082 -571140.553932508;-0.0004 -5.16221666799046e-09 500968.841789116 -563650.492974617;-0.00036 -5.03496212359846e-09 509411.244984698 -556032.262755338;-0.00032 -4.90656267223922e-09 517737.812456147 -548287.595594527;-0.00028 -4.77704751084071e-09 525946.650813823 -540418.252562708;-0.00024 -4.64644609003373e-09 534035.893438675 -532426.023080625;-0.0002 -4.51478810745513e-09 542003.700906689 -524312.72451234;-0.00016 -4.38210350099476e-09 549848.261407157 -516080.201751981;-0.00012 -4.24842244198792e-09 557567.791154671 -507730.32680423;-8e-05 -4.11377532835461e-09 565160.534794736 -499264.998358643;-4e-05 -3.97819277768732e-09 572624.765802925 -490686.141357908]  x2=[-0.00124 -2.14018094065136e-08 180354.238076816 -744261.886570259;-0.0012 -2.10755944278769e-08 191556.539517419 -741457.673804137;-0.00116 -2.07445870408154e-08 202715.282652848 -738484.85995705;-0.00112 -2.04088625135545e-08 213827.930081144 -735344.121021232;-0.00108 -2.00684971869566e-08 224891.954882113 -732036.171173631;-0.00104 -1.97235684571617e-08 235904.841191927 -728561.762613516;-0.001 -1.93741547579884e-08 246864.084775211 -724921.685391432;-0.00096 -1.90203355430988e-08 257767.193594483 -721116.767229548;-0.00092 -1.86621912679311e-08 268611.688376821 -717147.873333442;-0.00088 -1.82998033714049e-08 279395.10317763 -713015.90619536;-0.00084 -1.79332542574029e-08 290114.985941377 -708721.805388997;-0.0008 -1.75626272760325e-08 300768.899059167 -704266.547355845;-0.00076 -1.71880067046732e-08 311354.419923031 -699651.14518316;-0.00072 -1.68094777288123e-08 321869.141476811 -694876.648373595;-0.00068 -1.64271264226746e-08 332310.6727635 -689944.14260655;-0.00064 -1.604103972965e-08 342676.639468928 -684854.749491302;-0.0006 -1.56513054425228e-08 352964.684461658 -679609.626311956;-0.00056 -1.52580121835091e-08 363172.468328979 -674209.965764289;-0.00052 -1.48612493841044e-08 373297.669908868 -668656.995684548;-0.00048 -1.44611072647477e-08 383337.986817802 -662951.97877024;-0.00044 -1.40576768143063e-08 393291.1359743 -657096.212293014;-0.0004 -1.36510497693855e-08 403154.854118075 -651091.027803668;-0.00036 -1.32413185934689e-08 412926.898324684 -644937.790829371;-0.00032 -1.28285764558923e-08 422605.046515543 -638637.900563145;-0.00028 -1.24129172106586e-08 432187.097963215 -632192.78954571;-0.00024 -1.19944353750956e-08 441670.873791834 -625603.92333973;-0.0002 -1.1573226108364e-08 451054.217472559 -618872.800196562;-0.00016 -1.11493851898185e-08 460334.995313957 -612000.95071556;-0.00012 -1.07230089972291e-08 469511.096947181 -604989.937496038;-8e-05 -1.0294194484865e-08 478580.43580585 -597841.35478194;-4e-05 -9.8630391614484e-09 487540.949600518 -590556.828099328]  x3=[-0.00124 -1.83295585513564e-10 -23.6726386119881 -3420.16154076194;-0.0012 -1.84327359428236e-10 27.9029281941241 -3420.12966740018;-0.00116 -1.85317218890945e-10 79.4721501149895 -3419.320086046;-0.00112 -1.86264938816186e-10 131.023300754258 -3417.73298079121;-0.00108 -1.8717030370062e-10 182.544657824831 -3415.36871252987;-0.00104 -1.88033107672081e-10 234.024505814413 -3412.22781887618;-0.001 -1.88853154536386e-10 285.451138649513 -3408.31101404228;-0.00096 -1.89630257821949e-10 336.812862357312 -3403.6191886758;-0.00092 -1.90364240822186e-10 388.09799772476 -3398.15340965739;-0.00088 -1.91054936635691e-10 439.29488295434 -3391.91491985804;-0.00084 -1.91702188204192e-10 490.391876315854 -3384.90513785655;-0.0008 -1.92305848348265e-10 541.377358793654 -3377.12565761688;-0.00076 -1.92865779800799e-10 592.239736728703 -3368.57824812577;-0.00072 -1.9338185523821e-10 642.967444454878 -3359.26485299041;-0.00068 -1.93853957309393e-10 693.548946928899 -3349.18758999655;-0.00064 -1.9428197866241e-10 743.9727423533 -3338.34875062689;-0.0006 -1.94665821968895e-10 794.227364791838 -3326.75079954003;-0.00056 -1.95005399946191e-10 844.301386776747 -3314.39637401004;-0.00052 -1.95300635377195e-10 894.183421907248 -3301.28828332672;-0.00048 -1.95551461127914e-10 943.862127438716 -3287.42950815688;-0.00044 -1.95757820162737e-10 993.326206861925 -3272.82319986647;-0.0004 -1.95919665557399e-10 1042.56441247177 -3257.47267980403;-0.00036 -1.96036960509652e-10 1091.56554792492 -3241.38143854546;-0.00032 -1.96109678347636e-10 1140.31847078573 -3224.55313510024;-0.00028 -1.96137802535941e-10 1188.81209505997 -3206.99159607946;-0.00024 -1.9612132667937e-10 1237.03539371567 -3188.70081482565;-0.0002 -1.96060254524391e-10 1284.97740119058 -3169.68495050473;-0.00016 -1.95954599958284e-10 1332.62721588563 -3149.94832716027;-0.00012 -1.95804387005987e-10 1379.97400264388 -3129.49543273021;-8e-05 -1.95609649824631e-10 1427.00699521431 -3108.33091802637;-4e-05 -1.9537043269577e-10 1473.71549870002 -3086.45959567687]  x4=[-0.00124 5.1466373679587e-11 3052.8692706168 -13125.6249452388;-0.0012 5.36503492493801e-11 3250.44503709154 -13078.0977428376;-0.00116 5.58221251924148e-11 3447.28168039549 -13027.5966937905;-0.00112 5.79812076655702e-11 3643.33444157341 -12974.1332816003;-0.00108 6.01271057121111e-11 3838.55873991808 -12917.7196633861;-0.00104 6.22593313733271e-11 4032.91018310763 -12858.3686671181;-0.001 6.43773997994905e-11 4226.34457729987 -12796.0937887011;-0.00096 6.64808293601065e-11 4418.81793718167 -12730.9091889053;-0.00092 6.85691417534323e-11 4610.28649597083 -12662.8296901467;-0.00088 7.06418621152384e-11 4800.70671536822 -12591.870773116;-0.00084 7.2698519126789e-11 4990.03529545806 -12518.0485732593;-0.0008 7.47386451220155e-11 5178.22918455395 -12441.3798771081;-0.00076 7.67617761938599e-11 5365.24558898842 -12361.8821184627;-0.00072 7.87674522997632e-11 5551.04198284386 -12279.5733744278;-0.00068 8.0755217366275e-11 5735.57611762254 -12194.4723613022;-0.00064 8.27246193927612e-11 5918.80603185359 -12106.5984303223;-0.0006 8.46752105541841e-11 6100.69006063459 -12015.9715632621;-0.00056 8.66065473029349e-11 6281.18684510592 -11922.6123678898;-0.00052 8.85181904696921e-11 6460.25534185533 -11826.5420732813;-0.00048 9.04097053632849e-11 6637.85483225086 -11727.7825249931;-0.00044 9.22806618695381e-11 6813.94493169996 -11626.3561800947;-0.0004 9.41306345490768e-11 6988.48559883255 -11522.2861020625;-0.00036 9.5959202734067e-11 7161.4371446061 -11415.5959555346;-0.00032 9.77659506238724e-11 7332.76024133057 -11306.3100009303;-0.00028 9.95504673796035e-11 7502.41593161119 -11194.4530889333;-0.00024 1.01312347217539e-10 7670.36563720705 -11080.0506548407;-0.0002 1.03051189501398e-10 7836.57116780342 -10963.1287127794;-0.00016 1.0476659883344e-10 8000.99472969594 -10843.7138497909;-0.00012 1.06458185144376e-10 8163.59893438457 -10721.8332197852;-8e-05 1.08125563782066e-10 8324.3468070754 -10597.5145373664;-4e-05 1.09768355598988e-10 8483.20179508841 -10470.7860715309]  x5=0.00123288061605072  V1=ones(3,3)  V2=ones(3,3)  I1=ones(3,3)  I2=ones(3,3)  nHarmo=1  Measurements=None  Decoupling=off  VsMag0=0  VrMag0=0  VsAngle0=0  VrAngle0=0  IsMag0=0  IrMag0=0  IsAngle0=0  IrAngle0=0
      settings: AttributesFormatString=\n
  LMO7 : powerlib/Measurements/Three-Phase V-I Measurement  VoltageMeasurement=no  SetLabelV=on  LabelV=Vabc_LMO7  Vpu=on  VpuLL=off  CurrentMeasurement=no  SetLabelI=off  LabelI=A1  Ipu=off  Pbase=100e6  Vbase=735e3  OutputType=Magnitude  PhasorSimulation=off  PSBequivalent=0
  LVD 990 Mvar : powerlib/Elements/Three-Phase Series RLC Load  LConnTagsString=A|B|C  Configuration=Y (grounded)  NominalVoltage=735e3  Vabc=[1e3 1e3 1e3]  Vabcp=[1e3 1e3 1e3]  NominalFrequency=60  UnbalancedPower=off  ActivePower=3300000  InductivePower=990e6  CapacitivePower=0  Pabc=[10e3 9e3 11e3]  QLabc=[100 90 110]  QCabc=[100 90 110]  Pabcp=[10e3 9e3 11e3]  QLabcp=[100 90 110]  QCabcp=[100 90 110]  Measurements=None  LoadType=constant Z
  LVD-MTL 3*260km : powerlib/Elements/Distributed Parameters Line  Phases=3  Length=260  Frequency=60  Resistance="[0.01273  0.3864]/3"  Inductance="[0.9337e-3  4.1264e-3]/3"  Capacitance=[12.74e-9 7.751e-9]*3  x1=[-0.00148 -7.54637943622753e-08 -29978.3042370811 -777966.187578071;-0.00144 -7.44939487513591e-08 -18243.8667891953 -778329.756012956;-0.0014 -7.35071638589053e-08 -6505.28084332991 -778516.338973354;-0.00136 -7.25036640712888e-08 5234.78434730007 -778525.894031909;-0.00132 -7.14836775757074e-08 16973.6591931123 -778358.419015882;-0.00128 -7.04474363082943e-08 28708.6743751987 -778013.952007648;-0.00124 -6.93951759013775e-08 40437.1614523052 -777492.571336034;-0.0012 -6.83271356298993e-08 52156.4534676126 -776794.395558508;-0.00116 -6.72435583570069e-08 63863.8855551796 -775919.583434222;-0.00112 -6.61446904788279e-08 75556.7955459101 -774868.333887909;-0.00108 -6.50307818684415e-08 87232.5245729075 -773640.885964649;-0.00104 -6.39020858190598e-08 98888.4176760782 -772237.518775516;-0.001 -6.2758858986431e-08 110521.824405847 -770658.551434106;-0.00096 -6.16013613304781e-08 122130.099425845 -768904.342983976;-0.00092 -6.0429856056186e-08 133710.603114439 -766975.292317001;-0.00088 -5.92446095537517e-08 145260.702164956 -764871.838082666;-0.00084 -5.80458913380086e-08 156777.770184476 -762594.458588324;-0.0008 -5.68339739871418e-08 168259.188291049 -760143.671690434;-0.00076 -5.56091330807055e-08 179702.345709211 -757520.034676802;-0.00072 -5.43716471369594e-08 191104.640363645 -754724.144139858;-0.00068 -5.31217975495355e-08 202463.479470877 -751756.635841001;-0.00064 -5.18598685234518e-08 213776.280128848 -748618.184566027;-0.0006 -5.05861470104862e-08 225040.469904246 -745309.503971691;-0.00056 -4.93009226439268e-08 236253.487417454 -741831.346423427;-0.00052 -4.80044876727112e-08 247412.782924986 -738184.502824267;-0.00048 -4.66971368949719e-08 258515.818899278 -734369.802434997;-0.00044 -4.53791675910017e-08 269560.070605698 -730388.112685589;-0.0004 -4.40508794556546e-08 280543.02667665 -726240.338977955;-0.00036 -4.27125745301978e-08 291462.189682635 -721927.424480068;-0.00032 -4.13645571336304e-08 302315.076700149 -717450.34991149;-0.00028 -4.00071337934836e-08 313099.219876275 -712810.133320372;-0.00024 -3.8640613176119e-08 323812.166989855 -708007.829851948;-0.0002 -3.72653060165405e-08 334451.482009098 -703044.531508616;-0.00016 -3.58815250477363e-08 345014.745645519 -697921.366901617;-0.00012 -3.44895849295652e-08 355499.555904061 -692639.500994402;-8e-05 -3.30898021772067e-08 365903.528629288 -687200.134837729;-4e-05 -3.16824950891874e-08 376224.298047522 -681604.505296556]  x2=[-0.00148 -1.08085064285749e-07 -239044.185522636 -695043.14179714;-0.00144 -1.06623391136847e-07 -228536.391891935 -698568.657558866;-0.0014 -1.05137472748281e-07 -217976.631056532 -701935.324832062;-0.00136 -1.03627647005079e-07 -207367.304214978 -705142.378065624;-0.00132 -1.02094257228595e-07 -196710.823836704 -708189.088003303;-0.00128 -1.00537652098441e-07 -186009.613113452 -711074.761849533;-0.00124 -9.89581855731986e-08 -175266.105408257 -713798.743426965;-0.0012 -9.73562168099365e-08 -164482.743702122 -716360.413325681;-0.00116 -9.5732110082536e-08 -153661.980038508 -718759.189044035;-0.00112 -9.40862346988613e-08 -142806.274965757 -720994.525121116;-0.00108 -9.24189649167812e-08 -131918.096977589 -723065.913260776;-0.00104 -9.07306798590662e-08 -120999.921951781 -724972.882447216;-0.001 -8.90217634271793e-08 -110054.23258718 -726714.999052087;-0.00096 -8.72926042139801e-08 -99083.5178391557 -728291.866933097;-0.00092 -8.5543595415362e-08 -88090.2723536348 -729703.127524088;-0.00088 -8.3775134740843e-08 -77076.9958998389 -730948.459916572;-0.00084 -8.19876243231299e-08 -66046.192801859 -732027.580932702;-0.0008 -8.01814706266769e-08 -55000.3713691942 -732940.245189664;-0.00076 -7.8357084355259e-08 -43942.043326383 -733686.245155478;-0.00072 -7.65148803585813e-08 -32873.7232418594 -734265.411196185;-0.00068 -7.46552775379464e-08 -21797.9279561615 -734677.61161442;-0.00064 -7.2778698750999e-08 -10717.1760096237 -734922.752679364;-0.0006 -7.08855707155724e-08 366.012930317724 -735000.778648053;-0.00056 -6.89763239126562e-08 11449.1186420751 -734911.671778054;-0.00052 -6.70513924885088e-08 22529.6209229862 -734655.452331502;-0.00048 -6.5111214155936e-08 33605.0001623868 -734232.178570487;-0.00044 -6.31562300947594e-08 44672.7379145475 -733641.946743815;-0.0004 -6.11868848514954e-08 55730.3174713477 -732884.891065111;-0.00036 -5.92036262382694e-08 66775.2244345527 -731961.18368231;-0.00032 -5.72069052309871e-08 77804.9472875664 -730871.034638503;-0.00028 -5.51971758667866e-08 88816.9779665281 -729614.691824183;-0.00024 -5.31748951407942e-08 99808.8124306252 -728192.440920872;-0.0002 -5.11405229022076e-08 110777.95123149 -726604.605336159;-0.00016 -4.909452174973e-08 121721.900081553 -724851.546130164;-0.00012 -4.70373569263797e-08 132638.170421223 -722933.661933432;-8e-05 -4.49694962136973e-08 143524.279984762 -720851.388856292;-4e-05 -4.28914098253762e-08 154377.753364733 -718605.200389683]  x3=[-0.00148 -6.24983086219141e-10 714.129665880783 -1454.19273706674;-0.00144 -6.25227225983399e-10 735.976496388136 -1443.25903908701;-0.0014 -6.25329194468198e-10 757.655972187 -1431.99715644793;-0.00136 -6.25288968486784e-10 779.163163551536 -1420.40965000449;-0.00132 -6.25106557186199e-10 800.493179931897 -1408.49915465574;-0.00128 -6.24782002045199e-10 821.641171066302 -1396.26837874559;-0.00124 -6.24315376864824e-10 842.602328083937 -1383.72010344702;-0.0012 -6.23706787751617e-10 863.371884598459 -1370.85718212962;-0.00116 -6.22956373093494e-10 883.945117791825 -1357.68253971078;-0.00112 -6.22064303528275e-10 904.317349488223 -1344.19917199056;-0.00108 -6.21030781904889e-10 924.483947217849 -1330.41014497051;-0.00104 -6.19856043237239e-10 944.440325270287 -1316.31859415646;-0.001 -6.18540354650768e-10 964.181945737265 -1301.92772384555;-0.00096 -6.17084015321713e-10 983.704319544534 -1287.24080639758;-0.00092 -6.15487356409081e-10 1003.00300747264 -1272.26118149093;-0.00088 -6.13750740979338e-10 1022.07362116638 -1256.99225536312;-0.00084 -6.11874563923857e-10 1040.91182413266 -1241.43750003628;-0.0008 -6.09859251869122e-10 1059.51333272656 -1225.60045252764;-0.00076 -6.07705263079713e-10 1077.87391712546 -1209.48471404522;-0.00072 -6.05413087354108e-10 1095.98940229079 -1193.09394916897;-0.00068 -6.02983245913298e-10 1113.85566891746 -1176.43188501749;-0.00064 -6.00416291282273e-10 1131.46865437049 -1159.50231040047;-0.0006 -5.97712807164381e-10 1148.82435360889 -1142.30907495719;-0.00056 -5.94873408308595e-10 1165.91882009632 -1124.85608828112;-0.00052 -5.91898740369729e-10 1182.74816669851 -1107.14731903092;-0.00048 -5.88789479761621e-10 1199.30856656718 -1089.186794028;-0.00044 -5.85546333503319e-10 1215.59625401021 -1070.97859734087;-0.0004 -5.82170039058315e-10 1231.60752534794 -1052.52686935643;-0.00036 -5.7866136416685e-10 1247.33873975533 -1033.8358058385;-0.00032 -5.75021106671336e-10 1262.78632008989 -1014.90965697374;-0.00028 -5.71250094334936e-10 1277.94675370507 -995.752726405201;-0.00024 -5.67349184653335e-10 1292.816593249 -976.369370253679;-0.0002 -5.63319264659755e-10 1307.3924574484 -956.763996127212;-0.00016 -5.5916125072325e-10 1321.67103187745 -936.941062118808;-0.00012 -5.54876088340332e-10 1335.64906971146 -916.905075792713;-8e-05 -5.50464751919973e-10 1349.32339246516 -896.660593159435;-4e-05 -5.45928244562033e-10 1362.69089071548 -876.212217639745]  x4=[-0.00148 -2.30738571666591e-10 -6436.5939226488 -14213.0814008033;-0.00144 -2.24569117394979e-10 -6221.5419385314 -14308.5226427326;-0.0014 -2.18348598042674e-10 -6005.07522942947 -14400.7102500044;-0.00136 -2.12078428102131e-10 -5787.24301800593 -14489.6232599518;-0.00132 -2.05760033355925e-10 -5568.09483742715 -14575.2414545231;-0.00128 -1.99394850552532e-10 -5347.68052009954 -14657.5453648791;-0.00124 -1.92984327079632e-10 -5126.0501863381 -14736.5162758205;-0.0012 -1.8652992063498e-10 -4903.25423296946 -14812.136230043;-0.00116 -1.80033098894941e-10 -4679.3433218721 -14884.3880322212;-0.00112 -1.73495339180752e-10 -4454.36836845629 -14953.2552529184;-0.00108 -1.66918128122594e-10 -4228.38053008633 -15018.7222323225;-0.00104 -1.60302961321541e-10 -4001.43119444783 -15080.7740838069;-0.001 -1.53651343009478e-10 -3773.57196786258 -15139.3966973157;-0.00096 -1.46964785707047e-10 -3544.85466355374 -15194.5767425721;-0.00092 -1.40244809879717e-10 -3315.33128986393 -15246.3016721097;-0.00088 -1.3349294359204e-10 -3085.05403842901 -15294.5597241256;-0.00084 -1.26710722160184e-10 -2854.07527231012 -15339.3399251549;-0.0008 -1.19899687802816e-10 -2622.44751408681 -15380.632092566;-0.00076 -1.13061389290412e-10 -2390.22343391381 -15418.4268368762;-0.00072 -1.06197381593083e-10 -2157.45583754435 -15452.7155638866;-0.00068 -9.93092255269874e-11 -1924.19765432255 -15483.4904766362;-0.00064 -9.23984873994132e-11 -1690.50192514772 -15510.7445771754;-0.0006 -8.54667386526149e-11 -1456.42179041338 -15534.4716681567;-0.00056 -7.85155555064808e-11 -1222.01047792355 -15554.6663542443;-0.00052 -7.15465186001139e-11 -987.321290789205 -15571.3240433406;-0.00048 -6.45612126324081e-11 -752.407595307634 -15584.4409476309;-0.00044 -5.7561226001702e-11 -517.322808827377 -15594.0140844442;-0.0004 -5.054815044459e-11 -282.120387601594 -15600.0412769317;-0.00036 -4.35235806739755e-11 -46.8538146325727 -15602.5211545619;-0.00032 -3.64891140164471e-11 188.423412489846 -15601.4531534319;-0.00028 -2.94463500490601e-11 423.657793753158 -15596.837516396;-0.00024 -2.23968902356065e-11 658.79583888764 -15588.6752930103;-0.0002 -1.53423375624559e-11 893.784079529572 -15576.968339294;-0.00016 -8.28429617405019e-12 1128.56908137949 -15561.7193173074;-0.00012 -1.22437100813527e-12 1363.09745635266 -15542.9316945466;-8e-05 5.83583256918838e-12 1597.31587471911 -15520.609743155;-4e-05 1.28947091285119e-11 1831.17107723031 -15494.7585389518]  x5=0.00147040807418893  V1=ones(3,3)  V2=ones(3,3)  I1=ones(3,3)  I2=ones(3,3)  nHarmo=1  Measurements=None  Decoupling=off  VsMag0=0  VrMag0=0  VsAngle0=0  VrAngle0=0  IsMag0=0  IrMag0=0  IsAngle0=0  IrAngle0=0
      settings: AttributesFormatString=\n
  LVD7 : powerlib/Measurements/Three-Phase V-I Measurement  VoltageMeasurement=no  SetLabelV=on  LabelV=Vabc_LVD7  Vpu=on  VpuLL=off  CurrentMeasurement=no  SetLabelI=off  LabelI=A1  Ipu=off  Pbase=100e6  Vbase=735e3  OutputType=Magnitude  PhasorSimulation=off  PSBequivalent=0
  Load Flow Bus1 : powerlib/Measurements/Load Flow Bus  LConnTagsString=a  Phases=single  Connectors=on one side  ID=LG31_13.8  Vbase=13.8e3  Vref=1  Vangle=0  VLF=1  VLFb=1  VLFc=1  angleLF=2.13  angleLFb=0  angleLFc=0
      settings: AttributesFormatString=%<ID>\n%<Vbase>V\n%<VLF>pu\n%<angleLF>deg.
  Load Flow Bus10 : powerlib/Measurements/Load Flow Bus  LConnTagsString=a  Phases=single  Connectors=on one side  ID=LVD7  Vbase=735e3  Vref=1  Vangle=0  VLF=1.053  VLFb=1  VLFc=1  angleLF=-6.263  angleLFb=0  angleLFc=0
      settings: AttributesFormatString=%<ID>\n%<Vbase>V\n%<VLF>pu\n%<angleLF>deg.
  Load Flow Bus11 : powerlib/Measurements/Load Flow Bus  LConnTagsString=a  Phases=single  Connectors=on one side  ID=CHM7  Vbase=735e3  Vref=1  Vangle=0  VLF=1.055  VLFb=1  VLFc=1  angleLF=1.134  angleLFb=0  angleLFc=0
      settings: AttributesFormatString=%<ID>\n%<Vbase>V\n%<VLF>pu\n%<angleLF>deg.
  Load Flow Bus12 : powerlib/Measurements/Load Flow Bus  LConnTagsString=a  Phases=single  Connectors=on one side  ID=LG47  Vbase=735e3  Vref=1  Vangle=0  VLF=1.01  VLFb=1  VLFc=1  angleLF=23.62  angleLFb=0  angleLFc=0
      settings: AttributesFormatString=%<ID>\n%<Vbase>V\n%<VLF>pu\n%<angleLF>deg.
  Load Flow Bus2 : powerlib/Measurements/Load Flow Bus  LConnTagsString=a  Phases=single  Connectors=on one side  ID=LG3_13.8  Vbase=13.8e3  Vref=1  Vangle=0  VLF=1  VLFb=1  VLFc=1  angleLF=1.566  angleLFb=0  angleLFc=0
      settings: AttributesFormatString=%<ID>\n%<Vbase>V\n%<VLF>pu\n%<angleLF>deg.
  Load Flow Bus3 : powerlib/Measurements/Load Flow Bus  LConnTagsString=a  Phases=single  Connectors=on one side  ID=LG4_13.8  Vbase=13.8e3  Vref=1  Vangle=0  VLF=1  VLFb=1  VLFc=1  angleLF=-0.4067  angleLFb=0  angleLFc=0
      settings: AttributesFormatString=%<ID>\n%<Vbase>V\n%<VLF>pu\n%<angleLF>deg.
  Load Flow Bus4 : powerlib/Measurements/Load Flow Bus  LConnTagsString=a  Phases=single  Connectors=on one side  ID=LG2_13.8  Vbase=13.8e3  Vref=1  Vangle=0  VLF=1  VLFb=1  VLFc=1  angleLF=0  angleLFb=0  angleLFc=0
      settings: AttributesFormatString=%<ID>\n%<Vbase>V\n%<VLF>pu\n%<angleLF>deg.
  Load Flow Bus5 : powerlib/Measurements/Load Flow Bus  LConnTagsString=a  Phases=single  Connectors=on one side  ID=LG27  Vbase=735e3  Vref=1  Vangle=0  VLF=1.009  VLFb=1  VLFc=1  angleLF=24.74  angleLFb=0  angleLFc=0
      settings: AttributesFormatString=%<ID>\n%<Vbase>V\n%<VLF>pu\n%<angleLF>deg.
  Load Flow Bus6 : powerlib/Measurements/Load Flow Bus  LConnTagsString=a  Phases=single  Connectors=on one side  ID=LG37  Vbase=735e3  Vref=1  Vangle=0  VLF=0.9995  VLFb=1  VLFc=1  angleLF=26.29  angleLFb=0  angleLFc=0
      settings: AttributesFormatString=%<ID>\n%<Vbase>V\n%<VLF>pu\n%<angleLF>deg.
  Load Flow Bus7 : powerlib/Measurements/Load Flow Bus  LConnTagsString=a  Phases=single  Connectors=on one side  ID=LMO7  Vbase=735e3  Vref=1  Vangle=0  VLF=1.026  VLFb=1  VLFc=1  angleLF=20.27  angleLFb=0  angleLFc=0
      settings: AttributesFormatString=%<ID>\n%<Vbase>V\n%<VLF>pu\n%<angleLF>deg.
  Load Flow Bus8 : powerlib/Measurements/Load Flow Bus  LConnTagsString=a  Phases=single  Connectors=on one side  ID=NEM_ALB7  Vbase=735e3  Vref=1  Vangle=0  VLF=1.043  VLFb=1  VLFc=1  angleLF=12.43  angleLFb=0  angleLFc=0
      settings: AttributesFormatString=%<ID>\n%<Vbase>V\n%<VLF>pu\n%<angleLF>deg.
  Load Flow Bus9 : powerlib/Measurements/Load Flow Bus  LConnTagsString=a  Phases=single  Connectors=on one side  ID=ABI_CHB7  Vbase=735e3  Vref=1  Vangle=0  VLF=1.059  VLFb=1  VLFc=1  angleLF=4.701  angleLFb=0  angleLFc=0
      settings: AttributesFormatString=%<ID>\n%<Vbase>V\n%<VLF>pu\n%<angleLF>deg.
  NEM-ABI 6*236 : powerlib/Elements/Distributed Parameters Line  Phases=3  Length=236  Frequency=60  Resistance="[0.01273  0.3864]/6"  Inductance="[0.9337e-3  4.1264e-3]/6"  Capacitance=[12.74e-9 7.751e-9]*6  x1=[-0.00136 -2.22826021974938e-08 0 0;-0.00132 -2.1980201233235e-08 0 0;-0.00128 -2.16728021607649e-08 0 0;-0.00124 -2.13604748799818e-08 0 0;-0.0012 -2.10432904114158e-08 0 0;-0.00116 -2.07213208800799e-08 0 0;-0.00112 -2.0394639499069e-08 0 0;-0.00108 -2.00633205529118e-08 0 0;-0.00104 -1.97274393806796e-08 0 0;-0.001 -1.93870723588544e-08 0 0;-0.00096 -1.90422968839618e-08 0 0;-0.00092 -1.86931913549716e-08 0 0;-0.00088 -1.83398351554704e-08 0 0;-0.00084 -1.7982308635611e-08 315441.409430803 -699073.961425471;-0.0008 -1.76206930938406e-08 325946.963479199 -694237.903107612;-0.00076 -1.7255070758415e-08 336378.399998947 -689243.981077439;-0.00072 -1.68855247687004e-08 346733.346971338 -684093.330909756;-0.00068 -1.65121391562679e-08 357009.449770729 -678787.123817994;-0.00064 -1.6134998825786e-08 367204.371699961 -673326.566387886;-0.0006 -1.57541895357133e-08 377315.794521704 -667712.900303103;-0.00056 -1.53697978787986e-08 387341.418985605 -661947.402062901;-0.00052 -1.49819112623897e-08 397278.965351119 -656031.382691862;-0.00048 -1.45906178885583e-08 407126.173905901 -649966.187441773;-0.00044 -1.41960067340431e-08 416880.805479642 -643753.195485728;-0.0004 -1.37981675300177e-08 426540.641953245 -637393.819604522;-0.00036 -1.33971907416864e-08 436103.486763197 -630889.505865387;-0.00032 -1.29931675477129e-08 445567.165401055 -624241.733293178;-0.00028 -1.25861898194873e-08 454929.525907909 -617452.01353405;-0.00024 -1.21763501002354e-08 464188.439363717 -610521.890511724;-0.0002 -1.17637415839751e-08 473341.800371404 -603452.940076411;-0.00016 -1.13484580943248e-08 482387.527535612 -596246.769646482;-0.00012 -1.09305940631688e-08 491323.563935992 -588905.017842949;-8e-05 -1.05102445091842e-08 500147.877594926 -581429.354116858;-4e-05 -1.00875050162348e-08 508858.461939587 -573821.478369674]  x2=[-0.00136 -3.66000970283275e-08 0 0;-0.00132 -3.60771565287639e-08 0 0;-0.00128 -3.55460123949219e-08 0 0;-0.00124 -3.5006785404397e-08 0 0;-0.0012 -3.44595981727568e-08 0 0;-0.00116 -3.3904575125659e-08 0 0;-0.00112 -3.33418424705583e-08 0 0;-0.00108 -3.27715281680075e-08 0 0;-0.00104 -3.2193761902561e-08 0 0;-0.001 -3.1608675053285e-08 0 0;-0.00096 -3.10164006638835e-08 0 0;-0.00092 -3.04170734124451e-08 0 0;-0.00088 -2.98108295808184e-08 0 0;-0.00084 -2.91978070236226e-08 177812.618117985 -753237.160913972;-0.0008 -2.85781451369008e-08 189150.545920726 -750470.251306362;-0.00076 -2.79519848264224e-08 200445.462520489 -747532.691235386;-0.00072 -2.7319468475642e-08 211694.799550643 -744425.148676869;-0.00068 -2.66807399133233e-08 222895.999008958 -741148.330259193;-0.00064 -2.60359443808333e-08 234046.513839271 -737702.981102607;-0.0006 -2.53852284991155e-08 245143.808510668 -734089.884649797;-0.00056 -2.47287402353498e-08 256185.35959404 -730309.86248774;-0.00052 -2.40666288693062e-08 267168.656335889 -726363.774160877;-0.00048 -2.33990449593995e-08 278091.201229252 -722252.516975665;-0.00044 -2.27261403084539e-08 288950.510581611 -717977.025796532;-0.0004 -2.20480679291839e-08 299744.115079667 -713538.272833304;-0.00036 -2.13649820094013e-08 310469.560350837 -708937.267420125;-0.00032 -2.06770378769535e-08 321124.407521359 -704175.055785949;-0.00028 -1.99843919644037e-08 331706.23377087 -699252.720816635;-0.00024 -1.92872017734592e-08 342212.632883333 -694171.381808706;-0.0002 -1.85856258391572e-08 352641.215794196 -688932.194214832;-0.00016 -1.7879823693815e-08 362989.611133634 -683536.349381092;-0.00012 -1.71699558307538e-08 373255.465765791 -677985.07427607;-8e-05 -1.64561836678041e-08 383436.44532385 -672279.631211851;-4e-05 -1.57386695106005e-08 393530.234740857 -666421.317556988]  x3=[-0.00136 -4.78518524004471e-10 0 0;-0.00132 -4.79302959150942e-10 0 0;-0.00128 -4.79978404937834e-10 0 0;-0.00124 -4.80544707774601e-10 0 0;-0.0012 -4.81001738888861e-10 0 0;-0.00116 -4.8134939435568e-10 0 0;-0.00112 -4.81587595121203e-10 0 0;-0.00108 -4.8171628702063e-10 0 0;-0.00104 -4.81735440790533e-10 0 0;-0.001 -4.8164505207551e-10 0 0;-0.00096 -4.81445141429175e-10 0 0;-0.00092 -4.81135754309484e-10 0 0;-0.00088 -4.80716961068402e-10 0 0;-0.00084 -4.80188856935899e-10 247.453736713545 -6549.88779586482;-0.0008 -4.79551561998302e-10 346.191896446366 -6545.41168534684;-0.00076 -4.78805221170982e-10 444.851335127367 -6539.44720465683;-0.00072 -4.77950004165409e-10 543.409618450995 -6531.99571006628;-0.00068 -4.76986105450554e-10 641.844335113552 -6523.05889598079;-0.00064 -4.75913744208672e-10 740.133101909334 -6512.63879455481;-0.0006 -4.74733164285463e-10 838.253568820377 -6500.73777522956;-0.00056 -4.73444634134619e-10 936.183424098662 -6487.3585441942;-0.00052 -4.72048446756786e-10 1033.90039933961 -6472.50414377048;-0.00048 -4.70544919632933e-10 1131.38227454572 -6456.17795172098;-0.00044 -4.68934394652162e-10 1228.60688317923 -6438.38368048095;-0.0004 -4.67217238033965e-10 1325.55211720256 -6419.12537631424;-0.00036 -4.65393840244949e-10 1422.19593210551 -6398.40741839314;-0.00032 -4.63464615910047e-10 1518.51635191799 -6376.23451780261;-0.00028 -4.61430003718235e-10 1614.49147420718 -6352.61171646904;-0.00024 -4.59290466322781e-10 1710.09947505791 -6327.54438601373;-0.0002 -4.57046490236037e-10 1805.31861403529 -6301.03822653146;-0.00016 -4.54698585718815e-10 1900.12723912823 -6273.09926529432;-0.00012 -4.52247286664354e-10 1994.503791673 -6243.73385538115;-8e-05 -4.4969315047692e-10 2088.42681125541 -6212.94867423294;-4e-05 -4.47036757945056e-10 2181.87494059077 -6180.75072213439]  x4=[-0.00136 -7.59827194708808e-11 0 0;-0.00132 -7.06757720668462e-11 0 0;-0.00128 -6.53527536017254e-11 0 0;-0.00124 -6.00148744840138e-11 0 0;-0.0012 -5.46633485013908e-11 0 0;-0.00116 -4.92993925447151e-11 0 0;-0.00112 -4.39242263313147e-11 0 0;-0.00108 -3.85390721276329e-11 0 0;-0.00104 -3.31451544712962e-11 0 0;-0.001 -2.77436998926642e-11 0 0;-0.00096 -2.23359366359282e-11 0 0;-0.00092 -1.6923094379818e-11 0 0;-0.00088 -1.15064039579844e-11 0 0;-0.00084 -6.08709707911783e-12 5643.26911008038 -27050.3840473205;-0.0008 -6.66406046868327e-13 6050.52329986988 -26962.2123954925;-0.00076 4.7544365203694e-12 6456.40165283848 -26867.909769078;-0.00072 1.01741979697429e-11 6860.81187574886 -26767.497611681;-0.00068 1.55916458942366e-11 7263.66200920381 -26660.9987561601;-0.00064 2.10055484129107e-11 7664.86044855703 -26548.4374194368;-0.0006 2.64146744510197e-11 8064.31596474318 -26429.8391969883;-0.00056 3.18177940199491e-11 8461.93772502266 -26305.2310570275;-0.00052 3.72136784969032e-11 8857.6353136361 -26174.6413343711;-0.00048 4.26011009042843e-11 9251.31875236422 -26038.0997239957;-0.00044 4.7978836188696e-11 9642.89852098802 -25895.6372742861;-0.0004 5.33456614995102e-11 10032.285577645 -25747.2863799748;-0.00036 5.87003564669329e-11 10419.3913790763 -25593.0807747759;-0.00032 6.40417034795053e-11 10804.127900761 -25433.055523714;-0.00028 6.93684879609785e-11 11186.407656932 -25267.2470151514;-0.00024 7.46794986464978e-11 11566.1437204692 -25095.692952513;-0.0002 7.99735278580335e-11 11943.2497426666 -24918.4323457133;-0.00016 8.52493717789966e-11 12317.6399728666 -24735.5055022855;-0.00012 9.05058307279764e-11 12689.2292779597 -24546.9540182165;-8e-05 9.57417094315377e-11 13057.9331617422 -24352.8207684876;-4e-05 1.00955817296016e-10 13423.6677841305 -24153.1498973258]  x5=0.00133467809810995  V1=ones(3,3)  V2=ones(3,3)  I1=ones(3,3)  I2=ones(3,3)  nHarmo=1  Measurements=None  Decoupling=off  VsMag0=0  VrMag0=0  VsAngle0=0  VrAngle0=0  IsMag0=0  IrMag0=0  IsAngle0=0  IrAngle0=0
      settings: AttributesFormatString=\n
  NEM-ALB 1980 Mvar : powerlib/Elements/Three-Phase Series RLC Load  LConnTagsString=A|B|C  Configuration=Y (grounded)  NominalVoltage=735e3  Vabc=[1e3 1e3 1e3]  Vabcp=[1e3 1e3 1e3]  NominalFrequency=60  UnbalancedPower=off  ActivePower=6600000  InductivePower=1980e6  CapacitivePower=0  Pabc=[10e3 9e3 11e3]  QLabc=[100 90 110]  QCabc=[100 90 110]  Pabcp=[10e3 9e3 11e3]  QLabcp=[100 90 110]  QCabcp=[100 90 110]  Measurements=None  LoadType=constant Z
  NEM-ALB7 : powerlib/Measurements/Three-Phase V-I Measurement  VoltageMeasurement=no  SetLabelV=on  LabelV=Vabc_NEM7  Vpu=on  VpuLL=off  CurrentMeasurement=no  SetLabelI=off  LabelI=A1  Ipu=off  Pbase=100e6  Vbase=735e3  OutputType=Magnitude  PhasorSimulation=off  PSBequivalent=0
  Regulators1 : Subsystem
  Regulators2 : Subsystem
  Regulators3 : Subsystem
  Regulators4 : Subsystem
  MTLa : PMIOPort  Side=Right
  MTLb : PMIOPort  Port=2  Side=Right
  MTLc : PMIOPort  Port=3  Side=Right
  CHM7a : PMIOPort  Port=4  Side=Right
  CHM7b : PMIOPort  Port=5  Side=Right
  CHM7c : PMIOPort  Port=6  Side=Right
  wires:
  Regulators2/1(Pm) -> LG3_2200 MVA/1
  Regulators4/2(Vf) -> LG4-2700 MVA/2
  Regulators4/1(Pm) -> LG4-2700 MVA/1
  Regulators3/2(Vf) -> LG31-200 MVA/2
  Regulators3/1(Pm) -> LG31-200 MVA/1
  Regulators2/2(Vf) -> LG3_2200 MVA/2
  LG3_2200 MVA/1 -> Regulators2/1(m)
  Regulators1/1(Pm) -> LG2_5500 MVA/1
  Regulators1/2(Vf) -> LG2_5500 MVA/2
  LG2_5500 MVA/1 -> Regulators1/1(m)
  LG31-200 MVA/1 -> Regulators3/1(m)
  LG4-2700 MVA/1 -> Regulators4/1(m)
  connections:
  LG2-NENI 3*279km/RConn1 -- "Cs NEM "/LConn1
  LG2-NENI 3*279km/RConn2 -- "Cs NEM "/LConn2
  LG2-NENI 3*279km/RConn3 -- "Cs NEM "/LConn3
  CHB-CHM 3*195km/RConn1 -- "Cs  CHMN "/LConn1
  CHB-CHM 3*195km/RConn2 -- "Cs  CHMN "/LConn2
  CHB-CHM 3*195km/RConn3 -- "Cs  CHMN "/LConn3
  Load Flow Bus2/LConn1 -- 2200 MVA 13.8 kV/735 kV/LConn1 -- LG3_2200 MVA/RConn1 -- 110 MW/LConn1
  2200 MVA 13.8 kV/735 kV/LConn2 -- LG3_2200 MVA/RConn2 -- 110 MW/LConn2
  2200 MVA 13.8 kV/735 kV/LConn3 -- LG3_2200 MVA/RConn3 -- 110 MW/LConn3
  Load Flow Bus1/LConn1 -- 200 MVA 13.8 kV/735 kV/LConn1 -- LG31-200 MVA/RConn1 -- 10 MW/LConn1
  200 MVA 13.8 kV/735 kV/LConn2 -- LG31-200 MVA/RConn2 -- 10 MW/LConn2
  200 MVA 13.8 kV/735 kV/LConn3 -- LG31-200 MVA/RConn3 -- 10 MW/LConn3
  Load Flow Bus6/LConn1 -- 2200 MVA 13.8 kV/735 kV/RConn1 -- 200 MVA 13.8 kV/735 kV/RConn1 -- LG3-LMO 104km/LConn1 -- LG3 660 Mvar/LConn1 -- LG2-LG3 155km/RConn1
  2200 MVA 13.8 kV/735 kV/RConn2 -- LG3 660 Mvar/LConn2 -- LG2-LG3 155km/RConn2 -- 200 MVA 13.8 kV/735 kV/RConn2 -- LG3-LMO 104km/LConn2
  LG3-LMO 104km/RConn1 -- LMO7/RConn1 -- LG4-LMO 3*118km/RConn1 -- LMO 330 Mvar/LConn1
  LG3-LMO 104km/RConn2 -- LMO7/RConn2 -- LG4-LMO 3*118km/RConn2 -- LMO 330 Mvar/LConn2
  LG3-LMO 104km/RConn3 -- LMO7/RConn3 -- LG4-LMO 3*118km/RConn3 -- LMO 330 Mvar/LConn3
  LG4-LMO 3*118km/LConn1 -- LG4 660 Mvar/LConn1 -- 2700 MVA 13.8 kV/735 kV/RConn1 -- Load Flow Bus12/LConn1
  LG4-LMO 3*118km/LConn2 -- 2700 MVA 13.8 kV/735 kV/RConn2 -- LG4 660 Mvar/LConn2
  LG4 660 Mvar/LConn3 -- 2700 MVA 13.8 kV/735 kV/RConn3 -- LG4-LMO 3*118km/LConn3
  Load Flow Bus3/LConn1 -- LG4-2700 MVA/RConn1 -- 2700 MVA 13.8 kV/735 kV/LConn1 -- 135 MW/LConn1
  LG4-2700 MVA/RConn2 -- 2700 MVA 13.8 kV/735 kV/LConn2 -- 135 MW/LConn2
  LG4-2700 MVA/RConn3 -- 2700 MVA 13.8 kV/735 kV/LConn3 -- 135 MW/LConn3
  Load Flow Bus4/LConn1 -- 5500 MVA 13.8 kV/735 kV/LConn1 -- LG2_5500 MVA/RConn1 -- 275 MW/LConn1
  5500 MVA 13.8 kV/735 kV/LConn2 -- LG2_5500 MVA/RConn2 -- 275 MW/LConn2
  LG2_5500 MVA/RConn3 -- 5500 MVA 13.8 kV/735 kV/LConn3 -- 275 MW/LConn3
  5500 MVA 13.8 kV/735 kV/RConn1 -- LG2-NENI 3*279km/LConn1 -- LG2-LG3 155km/LConn1 -- LG2 660 Mvar/LConn1 -- Load Flow Bus5/LConn1
  LG2-LG3 155km/LConn2 -- 5500 MVA 13.8 kV/735 kV/RConn2 -- LG2-NENI 3*279km/LConn2 -- LG2 660 Mvar/LConn2
  LG2-LG3 155km/LConn3 -- 5500 MVA 13.8 kV/735 kV/RConn3 -- LG2-NENI 3*279km/LConn3 -- LG2 660 Mvar/LConn3
  "Cs NEM "/RConn1 -- NEM-ALB7/LConn1 -- Cs ALB/RConn1
  "Cs NEM "/RConn2 -- NEM-ALB7/LConn2 -- Cs ALB/RConn2
  "Cs NEM "/RConn3 -- NEM-ALB7/LConn3 -- Cs ALB/RConn3
  LMO7/LConn1 -- LMO-ALB 3*218km/LConn1
  LMO7/LConn2 -- LMO-ALB 3*218km/LConn2
  Load Flow Bus7/LConn1 -- LMO7/LConn3 -- LMO-ALB 3*218km/LConn3
  Cs ALB/LConn1 -- LMO-ALB 3*218km/RConn1
  Cs ALB/LConn2 -- LMO-ALB 3*218km/RConn2
  Cs ALB/LConn3 -- LMO-ALB 3*218km/RConn3
  200 MVA 13.8 kV/735 kV/RConn3 -- LG3-LMO 104km/LConn3 -- LG3 660 Mvar/LConn3 -- LG2-LG3 155km/RConn3 -- 2200 MVA 13.8 kV/735 kV/RConn3
  Load Flow Bus8/LConn1 -- NEM-ABI 6*236/LConn1 -- NEM-ALB7/RConn1 -- NEM-ALB 1980 Mvar/LConn1
  NEM-ALB 1980 Mvar/LConn2 -- NEM-ALB7/RConn2 -- NEM-ABI 6*236/LConn2
  NEM-ALB 1980 Mvar/LConn3 -- NEM-ALB7/RConn3 -- NEM-ABI 6*236/LConn3
  NEM-ABI 6*236/RConn1 -- "Cs ABI+CHB "/LConn1
  NEM-ABI 6*236/RConn2 -- "Cs ABI+CHB "/LConn2
  NEM-ABI 6*236/RConn3 -- "Cs ABI+CHB "/LConn3
  "Cs ABI+CHB "/RConn1 -- ABI-CHB7/LConn1
  "Cs ABI+CHB "/RConn2 -- ABI-CHB7/LConn2
  "Cs ABI+CHB "/RConn3 -- ABI-CHB7/LConn3
  Load Flow Bus9/LConn1 -- ABI+CHB 1320 Mvar/LConn1 -- CHB-CHM 3*195km/LConn1 -- ABI-CHB 3*271km/LConn1 -- ABI-CHB7/RConn1
  ABI-CHB 3*271km/LConn2 -- ABI-CHB7/RConn2 -- ABI+CHB 1320 Mvar/LConn2 -- CHB-CHM 3*195km/LConn2
  ABI-CHB 3*271km/LConn3 -- ABI-CHB7/RConn3 -- ABI+CHB 1320 Mvar/LConn3 -- CHB-CHM 3*195km/LConn3
  ABI-CHB 3*271km/RConn1 -- "Cs LVDN "/LConn1
  ABI-CHB 3*271km/RConn2 -- "Cs LVDN "/LConn2
  ABI-CHB 3*271km/RConn3 -- "Cs LVDN "/LConn3
  "Cs LVDN "/RConn1 -- LVD7/LConn1
  "Cs LVDN "/RConn2 -- LVD7/LConn2
  "Cs LVDN "/RConn3 -- LVD7/LConn3
  "Cs LVDS "/LConn1 -- LVD 990 Mvar/LConn1 -- Load Flow Bus10/LConn1 -- LVD7/RConn1
  "Cs LVDS "/LConn2 -- LVD7/RConn2 -- LVD 990 Mvar/LConn2
  "Cs LVDS "/LConn3 -- LVD7/RConn3 -- LVD 990 Mvar/LConn3
  "Cs LVDS "/RConn1 -- LVD-MTL 3*260km/LConn1
  "Cs LVDS "/RConn2 -- LVD-MTL 3*260km/LConn2
  "Cs LVDS "/RConn3 -- LVD-MTL 3*260km/LConn3
  MTLa/RConn1 -- LVD-MTL 3*260km/RConn1
  MTLb/RConn1 -- LVD-MTL 3*260km/RConn2
  MTLc/RConn1 -- LVD-MTL 3*260km/RConn3
  "Cs  CHMN "/RConn1 -- CHM7/LConn1
  "Cs  CHMN "/RConn2 -- CHM7/LConn2
  "Cs  CHMN "/RConn3 -- CHM7/LConn3
  CHM 1320Mvar/LConn2 -- CHM7/RConn2 -- CHM7b/RConn1
  Load Flow Bus11/LConn1 -- CHM 1320Mvar/LConn3 -- CHM7c/RConn1 -- CHM7/RConn3
  CHM7a/RConn1 -- CHM 1320Mvar/LConn1 -- CHM7/RConn1
